simulink library "IO"  (R2024a)
settings: Solver=VariableStepAuto  StartTime=0.0  StopTime=10.0  RelTol=1e-3
values from neighbouring files (symbols this model uses):
  ADCBits = 12.0    [IO.sldd]
  DigitalPolarity : value not decoded    [IO.sldd]
  Vref = 5.0    [IO.sldd]
undefined symbols (not defined in the file or in its folder): Bridge, dt, enum2Raptor, H, raptor_xcp_function
libraries: Raptor_lib x118, Utilities x27, Cooling x1
(part 3 of 4)

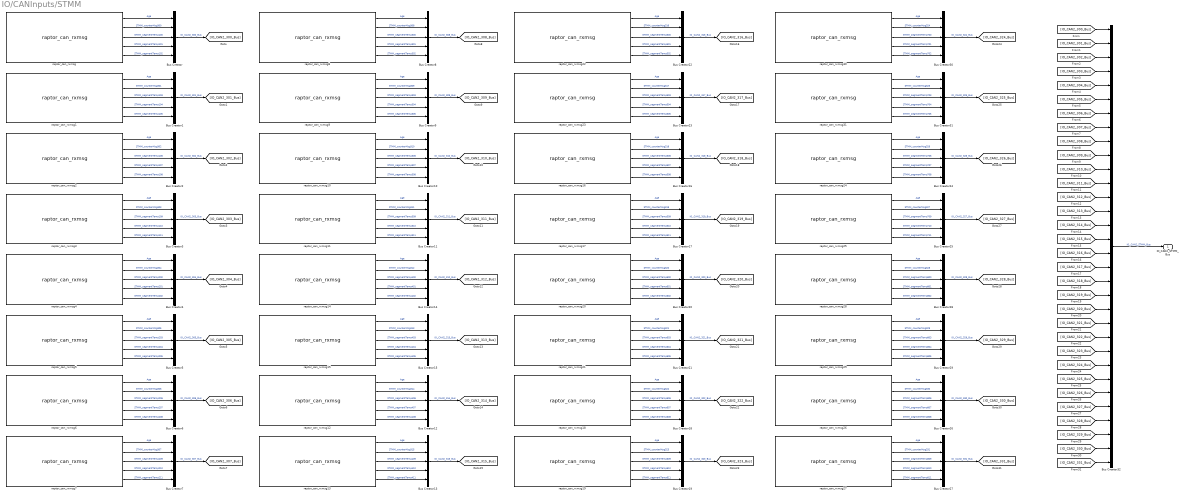
== system IO/CANInputs/STMM ==
  Bus Creator{,1..31} (32 alike) : BusCreator  Inputs=5
  Bus Creator32 : BusCreator  Inputs=32
  raptor_can_rxmsg : Raptor_lib/CAN/raptor_can_rxmsg  canDefinition=struct('dbcFile', 'raptor_CAN2.dbc','message', 'STMM_300','comment', '','signals', {{'STMM_counterMsg300','STMM_segmentTemp100','STMM_segmentTemp101','STMM_segmentTemp102'}},'enabled', [ 1 1 1 1;],'scaled', [ 1 1 1 1;],'canBus', '''CAN2''','messageID', [ 300;],'idMask', [ 536870911;],'payloadMask', [],'payloadValue', [],'period', [ 0;],'mailbox', '''''','queueSize', [ 1;],'label', [ 1;],'ver', [ 2;],'showID', [ 0;],'showRaw', [ 0;],'showRawMsg', [ 0;],'useStartVals', [ 0;],'extendedId', [ 0;],'showAge', [ 1;],'useSimFunc', [ 0;],'sim_func_name', '''''','fill', [ 0;],'editID', [ 0;],'signalOrder', [ 1;],'signalAscDes', [ 1;],'msgLength', [ 8;])  canBus='CAN2'  mailbox=''  payloadMask=[]  payloadValue=[]  idMask=hex2dec('1FFFFFFF')  queueSize=1  showID=0  label=1  fill=0  id=300  showRaw=0  showAge=1  signalOrder=1  signalInfo={{struct('Name', 'STMM_counterMsg300','StartBit', [ 0;],'SignalSize', [ 4;],'ByteOrder', 'LittleEndian','ValueType', 'UNSIGNED','Class', 'uint8','Signed', [ 0;],'Factor', [ 1;],'Offset', [ 0;],'Min', [ 0;],'Max', [ 15;],'Units', '','StartVal', [ 0;],'Comment', 'Counter Message 300','Multiplexed', [ 0;],'Multiplexor', [ 0;],'MultiplexMode_Min', [],'MultiplexMode_Max', []),struct('Name', 'STMM_segmentTemp100','StartBit', [ 16;],'SignalSize', [ 16;],'ByteOrder', 'LittleEndian','ValueType', 'SIGNED','Class', 'int16','Signed', [ 1;],'Factor', [ 0.1;],'Offset', [ 0;],'Min', [ -5;],'Max', [ 120;],'Units', 'degC','StartVal', [ 0;],'Comment', 'Segment 1 module 0','Multiplexed', [ 0;],'Multiplexor', [ 0;],'MultiplexMode_Min', [],'MultiplexMode_Max', []),struct('Name', 'STMM_segmentTemp101','StartBit', [ 32;],'SignalSize', [ 16;],'ByteOrder', 'LittleEndian','ValueType', 'SIGNED','Class', 'int16','Signed', [ 1;],'Factor', [ 0.1;],'Offset', [ 0;],'Min', [ -5;],'Max', [ 120;],'Units', 'degC','StartVal', [ 0;],'Comment', 'Segment 1 module 1','Multiplexed', [ 0;],'Multiplexor', [ 0;],'MultiplexMode_Min', [],'MultiplexMode_Max', []),struct('Name', 'STMM_segmentTemp102','StartBit', [ 48;],'SignalSize', [ 16;],'ByteOrder', 'LittleEndian','ValueType', 'SIGNED','Class', 'int16','Signed', [ 1;],'Factor', [ 0.1;],'Offset', [ 0;],'Min', [ -5;],'Max', [ 120;],'Units', 'degC','StartVal', [ 0;],'Comment', 'Segment 1 module 2','Multiplexed', [ 0;],'Multiplexor', [ 0;],'MultiplexMode_Min', [],'MultiplexMode_Max', [])}}  showRawMsg=0  useSimFunc=0  sim_func_name=''  useStartVals=0  extendedId=0
      settings: SourceProductName=Raptor
  raptor_can_rxmsg1 : Raptor_lib/CAN/raptor_can_rxmsg  canDefinition=struct('dbcFile', 'raptor_CAN2.dbc','message', 'STMM_301','comment', '','signals', {{'STMM_counterMsg301','STMM_segmentTemp103','STMM_segmentTemp104','STMM_segmentTemp105'}},'enabled', [ 1 1 1 1;],'scaled', [ 1 1 1 1;],'canBus', '''CAN2''','messageID', [ 301;],'idMask', [ 536870911;],'payloadMask', [],'payloadValue', [],'period', [ 0;],'mailbox', '''''','queueSize', [ 1;],'label', [ 1;],'ver', [ 2;],'showID', [ 0;],'showRaw', [ 0;],'showRawMsg', [ 0;],'useStartVals', [ 0;],'extendedId', [ 0;],'showAge', [ 1;],'useSimFunc', [ 0;],'sim_func_name', '''''','fill', [ 0;],'editID', [ 0;],'signalOrder', [ 1;],'signalAscDes', [ 1;],'msgLength', [ 8;])  canBus='CAN2'  mailbox=''  payloadMask=[]  payloadValue=[]  idMask=hex2dec('1FFFFFFF')  queueSize=1  showID=0  label=1  fill=0  id=301  showRaw=0  showAge=1  signalOrder=1  signalInfo={{struct('Name', 'STMM_counterMsg301','StartBit', [ 0;],'SignalSize', [ 4;],'ByteOrder', 'LittleEndian','ValueType', 'UNSIGNED','Class', 'uint8','Signed', [ 0;],'Factor', [ 1;],'Offset', [ 0;],'Min', [ 0;],'Max', [ 15;],'Units', '','StartVal', [ 0;],'Comment', 'Counter Message 301','Multiplexed', [ 0;],'Multiplexor', [ 0;],'MultiplexMode_Min', [],'MultiplexMode_Max', []),struct('Name', 'STMM_segmentTemp103','StartBit', [ 16;],'SignalSize', [ 16;],'ByteOrder', 'LittleEndian','ValueType', 'SIGNED','Class', 'int16','Signed', [ 1;],'Factor', [ 0.1;],'Offset', [ 0;],'Min', [ -5;],'Max', [ 120;],'Units', 'degC','StartVal', [ 0;],'Comment', 'Segment 1 module 3','Multiplexed', [ 0;],'Multiplexor', [ 0;],'MultiplexMode_Min', [],'MultiplexMode_Max', []),struct('Name', 'STMM_segmentTemp104','StartBit', [ 32;],'SignalSize', [ 16;],'ByteOrder', 'LittleEndian','ValueType', 'SIGNED','Class', 'int16','Signed', [ 1;],'Factor', [ 0.1;],'Offset', [ 0;],'Min', [ -5;],'Max', [ 120;],'Units', 'degC','StartVal', [ 0;],'Comment', 'Segment 1 module 4','Multiplexed', [ 0;],'Multiplexor', [ 0;],'MultiplexMode_Min', [],'MultiplexMode_Max', []),struct('Name', 'STMM_segmentTemp105','StartBit', [ 48;],'SignalSize', [ 16;],'ByteOrder', 'LittleEndian','ValueType', 'SIGNED','Class', 'int16','Signed', [ 1;],'Factor', [ 0.1;],'Offset', [ 0;],'Min', [ -5;],'Max', [ 120;],'Units', 'degC','StartVal', [ 0;],'Comment', 'Segment 1 module 5','Multiplexed', [ 0;],'Multiplexor', [ 0;],'MultiplexMode_Min', [],'MultiplexMode_Max', [])}}  showRawMsg=0  useSimFunc=0  sim_func_name=''  useStartVals=0  extendedId=0
      settings: SourceProductName=Raptor
  raptor_can_rxmsg10 : Raptor_lib/CAN/raptor_can_rxmsg  canDefinition=struct('dbcFile', 'raptor_CAN2.dbc','message', 'STMM_310','comment', '','signals', {{'STMM_counterMsg310','STMM_segmentTemp306','STMM_segmentTemp307','STMM_segmentTemp308'}},'enabled', [ 1 1 1 1;],'scaled', [ 1 1 1 1;],'canBus', '''CAN2''','messageID', [ 310;],'idMask', [ 536870911;],'payloadMask', [],'payloadValue', [],'period', [ 0;],'mailbox', '''''','queueSize', [ 1;],'label', [ 1;],'ver', [ 2;],'showID', [ 0;],'showRaw', [ 0;],'showRawMsg', [ 0;],'useStartVals', [ 0;],'extendedId', [ 0;],'showAge', [ 1;],'useSimFunc', [ 0;],'sim_func_name', '''''','fill', [ 0;],'editID', [ 0;],'signalOrder', [ 1;],'signalAscDes', [ 1;],'msgLength', [ 8;])  canBus='CAN2'  mailbox=''  payloadMask=[]  payloadValue=[]  idMask=hex2dec('1FFFFFFF')  queueSize=1  showID=0  label=1  fill=0  id=310  showRaw=0  showAge=1  signalOrder=1  signalInfo={{struct('Name', 'STMM_counterMsg310','StartBit', [ 0;],'SignalSize', [ 4;],'ByteOrder', 'LittleEndian','ValueType', 'UNSIGNED','Class', 'uint8','Signed', [ 0;],'Factor', [ 1;],'Offset', [ 0;],'Min', [ 0;],'Max', [ 15;],'Units', '','StartVal', [ 0;],'Comment', 'Counter Message 310','Multiplexed', [ 0;],'Multiplexor', [ 0;],'MultiplexMode_Min', [],'MultiplexMode_Max', []),struct('Name', 'STMM_segmentTemp306','StartBit', [ 16;],'SignalSize', [ 16;],'ByteOrder', 'LittleEndian','ValueType', 'SIGNED','Class', 'int16','Signed', [ 1;],'Factor', [ 0.1;],'Offset', [ 0;],'Min', [ -5;],'Max', [ 120;],'Units', 'degC','StartVal', [ 0;],'Comment', 'Segment 3 module 6','Multiplexed', [ 0;],'Multiplexor', [ 0;],'MultiplexMode_Min', [],'MultiplexMode_Max', []),struct('Name', 'STMM_segmentTemp307','StartBit', [ 32;],'SignalSize', [ 16;],'ByteOrder', 'LittleEndian','ValueType', 'SIGNED','Class', 'int16','Signed', [ 1;],'Factor', [ 0.1;],'Offset', [ 0;],'Min', [ -5;],'Max', [ 120;],'Units', 'degC','StartVal', [ 0;],'Comment', 'Segment 3 module 7','Multiplexed', [ 0;],'Multiplexor', [ 0;],'MultiplexMode_Min', [],'MultiplexMode_Max', []),struct('Name', 'STMM_segmentTemp308','StartBit', [ 48;],'SignalSize', [ 16;],'ByteOrder', 'LittleEndian','ValueType', 'SIGNED','Class', 'int16','Signed', [ 1;],'Factor', [ 0.1;],'Offset', [ 0;],'Min', [ -5;],'Max', [ 120;],'Units', 'degC','StartVal', [ 0;],'Comment', 'Segment 3 module 8','Multiplexed', [ 0;],'Multiplexor', [ 0;],'MultiplexMode_Min', [],'MultiplexMode_Max', [])}}  showRawMsg=0  useSimFunc=0  sim_func_name=''  useStartVals=0  extendedId=0
      settings: SourceProductName=Raptor
  raptor_can_rxmsg11 : Raptor_lib/CAN/raptor_can_rxmsg  canDefinition=struct('dbcFile', 'raptor_CAN2.dbc','message', 'STMM_311','comment', '','signals', {{'STMM_counterMsg311','STMM_segmentTemp309','STMM_segmentTemp310','STMM_segmentTemp311'}},'enabled', [ 1 1 1 1;],'scaled', [ 1 1 1 1;],'canBus', '''CAN2''','messageID', [ 311;],'idMask', [ 536870911;],'payloadMask', [],'payloadValue', [],'period', [ 0;],'mailbox', '''''','queueSize', [ 1;],'label', [ 1;],'ver', [ 2;],'showID', [ 0;],'showRaw', [ 0;],'showRawMsg', [ 0;],'useStartVals', [ 0;],'extendedId', [ 0;],'showAge', [ 1;],'useSimFunc', [ 0;],'sim_func_name', '''''','fill', [ 0;],'editID', [ 0;],'signalOrder', [ 1;],'signalAscDes', [ 1;],'msgLength', [ 8;])  canBus='CAN2'  mailbox=''  payloadMask=[]  payloadValue=[]  idMask=hex2dec('1FFFFFFF')  queueSize=1  showID=0  label=1  fill=0  id=311  showRaw=0  showAge=1  signalOrder=1  signalInfo={{struct('Name', 'STMM_segmentTemp311','StartBit', [ 48;],'SignalSize', [ 16;],'ByteOrder', 'LittleEndian','ValueType', 'SIGNED','Class', 'int16','Signed', [ 1;],'Factor', [ 0.1;],'Offset', [ 0;],'Min', [ -5;],'Max', [ 120;],'Units', 'degC','StartVal', [ 0;],'Comment', 'Segment 3 module 11','Multiplexed', [ 0;],'Multiplexor', [ 0;],'MultiplexMode_Min', [],'MultiplexMode_Max', []),struct('Name', 'STMM_segmentTemp310','StartBit', [ 32;],'SignalSize', [ 16;],'ByteOrder', 'LittleEndian','ValueType', 'SIGNED','Class', 'int16','Signed', [ 1;],'Factor', [ 0.1;],'Offset', [ 0;],'Min', [ -5;],'Max', [ 120;],'Units', 'degC','StartVal', [ 0;],'Comment', 'Segment 3 module 10','Multiplexed', [ 0;],'Multiplexor', [ 0;],'MultiplexMode_Min', [],'MultiplexMode_Max', []),struct('Name', 'STMM_segmentTemp309','StartBit', [ 16;],'SignalSize', [ 16;],'ByteOrder', 'LittleEndian','ValueType', 'SIGNED','Class', 'int16','Signed', [ 1;],'Factor', [ 0.1;],'Offset', [ 0;],'Min', [ -5;],'Max', [ 120;],'Units', 'degC','StartVal', [ 0;],'Comment', 'Segment 3 module 9','Multiplexed', [ 0;],'Multiplexor', [ 0;],'MultiplexMode_Min', [],'MultiplexMode_Max', []),struct('Name', 'STMM_counterMsg311','StartBit', [ 0;],'SignalSize', [ 4;],'ByteOrder', 'LittleEndian','ValueType', 'UNSIGNED','Class', 'uint8','Signed', [ 0;],'Factor', [ 1;],'Offset', [ 0;],'Min', [ 0;],'Max', [ 15;],'Units', '','StartVal', [ 0;],'Comment', 'Counter Message 311','Multiplexed', [ 0;],'Multiplexor', [ 0;],'MultiplexMode_Min', [],'MultiplexMode_Max', [])}}  showRawMsg=0  useSimFunc=0  sim_func_name=''  useStartVals=0  extendedId=0
      settings: SourceProductName=Raptor
  raptor_can_rxmsg12 : Raptor_lib/CAN/raptor_can_rxmsg  canDefinition=struct('dbcFile', 'raptor_CAN2.dbc','message', 'STMM_314','comment', '','signals', {{'STMM_counterMsg314','STMM_segmentTemp406','STMM_segmentTemp407','STMM_segmentTemp408'}},'enabled', [ 1 1 1 1;],'scaled', [ 1 1 1 1;],'canBus', '''CAN2''','messageID', [ 314;],'idMask', [ 536870911;],'payloadMask', [],'payloadValue', [],'period', [ 0;],'mailbox', '''''','queueSize', [ 1;],'label', [ 1;],'ver', [ 2;],'showID', [ 0;],'showRaw', [ 0;],'showRawMsg', [ 0;],'useStartVals', [ 0;],'extendedId', [ 0;],'showAge', [ 1;],'useSimFunc', [ 0;],'sim_func_name', '''''','fill', [ 0;],'editID', [ 0;],'signalOrder', [ 1;],'signalAscDes', [ 1;],'msgLength', [ 8;])  canBus='CAN2'  mailbox=''  payloadMask=[]  payloadValue=[]  idMask=hex2dec('1FFFFFFF')  queueSize=1  showID=0  label=1  fill=0  id=314  showRaw=0  showAge=1  signalOrder=1  signalInfo={{struct('Name', 'STMM_segmentTemp408','StartBit', [ 48;],'SignalSize', [ 16;],'ByteOrder', 'LittleEndian','ValueType', 'SIGNED','Class', 'int16','Signed', [ 1;],'Factor', [ 0.1;],'Offset', [ 0;],'Min', [ -5;],'Max', [ 120;],'Units', 'degC','StartVal', [ 0;],'Comment', 'Segment 4 module 8','Multiplexed', [ 0;],'Multiplexor', [ 0;],'MultiplexMode_Min', [],'MultiplexMode_Max', []),struct('Name', 'STMM_segmentTemp407','StartBit', [ 32;],'SignalSize', [ 16;],'ByteOrder', 'LittleEndian','ValueType', 'SIGNED','Class', 'int16','Signed', [ 1;],'Factor', [ 0.1;],'Offset', [ 0;],'Min', [ -5;],'Max', [ 120;],'Units', 'degC','StartVal', [ 0;],'Comment', 'Segment 4 module 7','Multiplexed', [ 0;],'Multiplexor', [ 0;],'MultiplexMode_Min', [],'MultiplexMode_Max', []),struct('Name', 'STMM_segmentTemp406','StartBit', [ 16;],'SignalSize', [ 16;],'ByteOrder', 'LittleEndian','ValueType', 'SIGNED','Class', 'int16','Signed', [ 1;],'Factor', [ 0.1;],'Offset', [ 0;],'Min', [ -5;],'Max', [ 120;],'Units', 'degC','StartVal', [ 0;],'Comment', 'Segment 4 module 6','Multiplexed', [ 0;],'Multiplexor', [ 0;],'MultiplexMode_Min', [],'MultiplexMode_Max', []),struct('Name', 'STMM_counterMsg314','StartBit', [ 0;],'SignalSize', [ 4;],'ByteOrder', 'LittleEndian','ValueType', 'UNSIGNED','Class', 'uint8','Signed', [ 0;],'Factor', [ 1;],'Offset', [ 0;],'Min', [ 0;],'Max', [ 15;],'Units', '','StartVal', [ 0;],'Comment', 'Counter Message 314','Multiplexed', [ 0;],'Multiplexor', [ 0;],'MultiplexMode_Min', [],'MultiplexMode_Max', [])}}  showRawMsg=0  useSimFunc=0  sim_func_name=''  useStartVals=0  extendedId=0
      settings: SourceProductName=Raptor
  raptor_can_rxmsg13 : Raptor_lib/CAN/raptor_can_rxmsg  canDefinition=struct('dbcFile', 'raptor_CAN2.dbc','message', 'STMM_315','comment', '','signals', {{'STMM_counterMsg315','STMM_segmentTemp409','STMM_segmentTemp410','STMM_segmentTemp411'}},'enabled', [ 1 1 1 1;],'scaled', [ 1 1 1 1;],'canBus', '''CAN2''','messageID', [ 315;],'idMask', [ 536870911;],'payloadMask', [],'payloadValue', [],'period', [ 0;],'mailbox', '''''','queueSize', [ 1;],'label', [ 1;],'ver', [ 2;],'showID', [ 0;],'showRaw', [ 0;],'showRawMsg', [ 0;],'useStartVals', [ 0;],'extendedId', [ 0;],'showAge', [ 1;],'useSimFunc', [ 0;],'sim_func_name', '''''','fill', [ 0;],'editID', [ 0;],'signalOrder', [ 1;],'signalAscDes', [ 1;],'msgLength', [ 8;])  canBus='CAN2'  mailbox=''  payloadMask=[]  payloadValue=[]  idMask=hex2dec('1FFFFFFF')  queueSize=1  showID=0  label=1  fill=0  id=315  showRaw=0  showAge=1  signalOrder=1  signalInfo={{struct('Name', 'STMM_segmentTemp411','StartBit', [ 48;],'SignalSize', [ 16;],'ByteOrder', 'LittleEndian','ValueType', 'SIGNED','Class', 'int16','Signed', [ 1;],'Factor', [ 0.1;],'Offset', [ 0;],'Min', [ -5;],'Max', [ 120;],'Units', 'degC','StartVal', [ 0;],'Comment', 'Segment 4 module 11','Multiplexed', [ 0;],'Multiplexor', [ 0;],'MultiplexMode_Min', [],'MultiplexMode_Max', []),struct('Name', 'STMM_segmentTemp410','StartBit', [ 32;],'SignalSize', [ 16;],'ByteOrder', 'LittleEndian','ValueType', 'SIGNED','Class', 'int16','Signed', [ 1;],'Factor', [ 0.1;],'Offset', [ 0;],'Min', [ -5;],'Max', [ 120;],'Units', 'degC','StartVal', [ 0;],'Comment', 'Segment 4 module 10','Multiplexed', [ 0;],'Multiplexor', [ 0;],'MultiplexMode_Min', [],'MultiplexMode_Max', []),struct('Name', 'STMM_segmentTemp409','StartBit', [ 16;],'SignalSize', [ 16;],'ByteOrder', 'LittleEndian','ValueType', 'SIGNED','Class', 'int16','Signed', [ 1;],'Factor', [ 0.1;],'Offset', [ 0;],'Min', [ -5;],'Max', [ 120;],'Units', 'degC','StartVal', [ 0;],'Comment', 'Segment 4 module 9','Multiplexed', [ 0;],'Multiplexor', [ 0;],'MultiplexMode_Min', [],'MultiplexMode_Max', []),struct('Name', 'STMM_counterMsg315','StartBit', [ 0;],'SignalSize', [ 4;],'ByteOrder', 'LittleEndian','ValueType', 'UNSIGNED','Class', 'uint8','Signed', [ 0;],'Factor', [ 1;],'Offset', [ 0;],'Min', [ 0;],'Max', [ 15;],'Units', '','StartVal', [ 0;],'Comment', 'Counter Message 315','Multiplexed', [ 0;],'Multiplexor', [ 0;],'MultiplexMode_Min', [],'MultiplexMode_Max', [])}}  showRawMsg=0  useSimFunc=0  sim_func_name=''  useStartVals=0  extendedId=0
      settings: SourceProductName=Raptor
  raptor_can_rxmsg14 : Raptor_lib/CAN/raptor_can_rxmsg  canDefinition=struct('dbcFile', 'raptor_CAN2.dbc','message', 'STMM_312','comment', '','signals', {{'STMM_counterMsg312','STMM_segmentTemp400','STMM_segmentTemp401','STMM_segmentTemp402'}},'enabled', [ 1 1 1 1;],'scaled', [ 1 1 1 1;],'canBus', '''CAN2''','messageID', [ 312;],'idMask', [ 536870911;],'payloadMask', [],'payloadValue', [],'period', [ 0;],'mailbox', '''''','queueSize', [ 1;],'label', [ 1;],'ver', [ 2;],'showID', [ 0;],'showRaw', [ 0;],'showRawMsg', [ 0;],'useStartVals', [ 0;],'extendedId', [ 0;],'showAge', [ 1;],'useSimFunc', [ 0;],'sim_func_name', '''''','fill', [ 0;],'editID', [ 0;],'signalOrder', [ 1;],'signalAscDes', [ 1;],'msgLength', [ 8;])  canBus='CAN2'  mailbox=''  payloadMask=[]  payloadValue=[]  idMask=hex2dec('1FFFFFFF')  queueSize=1  showID=0  label=1  fill=0  id=312  showRaw=0  showAge=1  signalOrder=1  signalInfo={{struct('Name', 'STMM_segmentTemp402','StartBit', [ 48;],'SignalSize', [ 16;],'ByteOrder', 'LittleEndian','ValueType', 'SIGNED','Class', 'int16','Signed', [ 1;],'Factor', [ 0.1;],'Offset', [ 0;],'Min', [ -5;],'Max', [ 120;],'Units', 'degC','StartVal', [ 0;],'Comment', 'Segment 4 module 2','Multiplexed', [ 0;],'Multiplexor', [ 0;],'MultiplexMode_Min', [],'MultiplexMode_Max', []),struct('Name', 'STMM_segmentTemp401','StartBit', [ 32;],'SignalSize', [ 16;],'ByteOrder', 'LittleEndian','ValueType', 'SIGNED','Class', 'int16','Signed', [ 1;],'Factor', [ 0.1;],'Offset', [ 0;],'Min', [ -5;],'Max', [ 120;],'Units', 'degC','StartVal', [ 0;],'Comment', 'Segment 4 module 1','Multiplexed', [ 0;],'Multiplexor', [ 0;],'MultiplexMode_Min', [],'MultiplexMode_Max', []),struct('Name', 'STMM_segmentTemp400','StartBit', [ 16;],'SignalSize', [ 16;],'ByteOrder', 'LittleEndian','ValueType', 'SIGNED','Class', 'int16','Signed', [ 1;],'Factor', [ 0.1;],'Offset', [ 0;],'Min', [ -5;],'Max', [ 120;],'Units', 'degC','StartVal', [ 0;],'Comment', 'Segment 4 module 0','Multiplexed', [ 0;],'Multiplexor', [ 0;],'MultiplexMode_Min', [],'MultiplexMode_Max', []),struct('Name', 'STMM_counterMsg312','StartBit', [ 0;],'SignalSize', [ 4;],'ByteOrder', 'LittleEndian','ValueType', 'UNSIGNED','Class', 'uint8','Signed', [ 0;],'Factor', [ 1;],'Offset', [ 0;],'Min', [ 0;],'Max', [ 15;],'Units', '','StartVal', [ 0;],'Comment', 'Counter Message 312','Multiplexed', [ 0;],'Multiplexor', [ 0;],'MultiplexMode_Min', [],'MultiplexMode_Max', [])}}  showRawMsg=0  useSimFunc=0  sim_func_name=''  useStartVals=0  extendedId=0
      settings: SourceProductName=Raptor
  raptor_can_rxmsg15 : Raptor_lib/CAN/raptor_can_rxmsg  canDefinition=struct('dbcFile', 'raptor_CAN2.dbc','message', 'STMM_313','comment', '','signals', {{'STMM_counterMsg313','STMM_segmentTemp403','STMM_segmentTemp404','STMM_segmentTemp405'}},'enabled', [ 1 1 1 1;],'scaled', [ 1 1 1 1;],'canBus', '''CAN2''','messageID', [ 313;],'idMask', [ 536870911;],'payloadMask', [],'payloadValue', [],'period', [ 0;],'mailbox', '''''','queueSize', [ 1;],'label', [ 1;],'ver', [ 2;],'showID', [ 0;],'showRaw', [ 0;],'showRawMsg', [ 0;],'useStartVals', [ 0;],'extendedId', [ 0;],'showAge', [ 1;],'useSimFunc', [ 0;],'sim_func_name', '''''','fill', [ 0;],'editID', [ 0;],'signalOrder', [ 1;],'signalAscDes', [ 1;],'msgLength', [ 8;])  canBus='CAN2'  mailbox=''  payloadMask=[]  payloadValue=[]  idMask=hex2dec('1FFFFFFF')  queueSize=1  showID=0  label=1  fill=0  id=313  showRaw=0  showAge=1  signalOrder=1  signalInfo={{struct('Name', 'STMM_segmentTemp405','StartBit', [ 48;],'SignalSize', [ 16;],'ByteOrder', 'LittleEndian','ValueType', 'SIGNED','Class', 'int16','Signed', [ 1;],'Factor', [ 0.1;],'Offset', [ 0;],'Min', [ -5;],'Max', [ 120;],'Units', 'degC','StartVal', [ 0;],'Comment', 'Segment 4 module 5','Multiplexed', [ 0;],'Multiplexor', [ 0;],'MultiplexMode_Min', [],'MultiplexMode_Max', []),struct('Name', 'STMM_segmentTemp404','StartBit', [ 32;],'SignalSize', [ 16;],'ByteOrder', 'LittleEndian','ValueType', 'SIGNED','Class', 'int16','Signed', [ 1;],'Factor', [ 0.1;],'Offset', [ 0;],'Min', [ -5;],'Max', [ 120;],'Units', 'degC','StartVal', [ 0;],'Comment', 'Segment 4 module 4','Multiplexed', [ 0;],'Multiplexor', [ 0;],'MultiplexMode_Min', [],'MultiplexMode_Max', []),struct('Name', 'STMM_segmentTemp403','StartBit', [ 16;],'SignalSize', [ 16;],'ByteOrder', 'LittleEndian','ValueType', 'SIGNED','Class', 'int16','Signed', [ 1;],'Factor', [ 0.1;],'Offset', [ 0;],'Min', [ -5;],'Max', [ 120;],'Units', 'degC','StartVal', [ 0;],'Comment', 'Segment 4 module 3','Multiplexed', [ 0;],'Multiplexor', [ 0;],'MultiplexMode_Min', [],'MultiplexMode_Max', []),struct('Name', 'STMM_counterMsg313','StartBit', [ 0;],'SignalSize', [ 4;],'ByteOrder', 'LittleEndian','ValueType', 'UNSIGNED','Class', 'uint8','Signed', [ 0;],'Factor', [ 1;],'Offset', [ 0;],'Min', [ 0;],'Max', [ 15;],'Units', '','StartVal', [ 0;],'Comment', 'Counter Message 313','Multiplexed', [ 0;],'Multiplexor', [ 0;],'MultiplexMode_Min', [],'MultiplexMode_Max', [])}}  showRawMsg=0  useSimFunc=0  sim_func_name=''  useStartVals=0  extendedId=0
      settings: SourceProductName=Raptor
  raptor_can_rxmsg16 : Raptor_lib/CAN/raptor_can_rxmsg  canDefinition=struct('dbcFile', 'raptor_CAN2.dbc','message', 'STMM_318','comment', '','signals', {{'STMM_counterMsg318','STMM_segmentTemp506','STMM_segmentTemp507','STMM_segmentTemp508'}},'enabled', [ 1 1 1 1;],'scaled', [ 1 1 1 1;],'canBus', '''CAN2''','messageID', [ 318;],'idMask', [ 536870911;],'payloadMask', [],'payloadValue', [],'period', [ 0;],'mailbox', '''''','queueSize', [ 1;],'label', [ 1;],'ver', [ 2;],'showID', [ 0;],'showRaw', [ 0;],'showRawMsg', [ 0;],'useStartVals', [ 0;],'extendedId', [ 0;],'showAge', [ 1;],'useSimFunc', [ 0;],'sim_func_name', '''''','fill', [ 0;],'editID', [ 0;],'signalOrder', [ 1;],'signalAscDes', [ 1;],'msgLength', [ 8;])  canBus='CAN2'  mailbox=''  payloadMask=[]  payloadValue=[]  idMask=hex2dec('1FFFFFFF')  queueSize=1  showID=0  label=1  fill=0  id=318  showRaw=0  showAge=1  signalOrder=1  signalInfo={{struct('Name', 'STMM_segmentTemp508','StartBit', [ 48;],'SignalSize', [ 16;],'ByteOrder', 'LittleEndian','ValueType', 'SIGNED','Class', 'int16','Signed', [ 1;],'Factor', [ 0.1;],'Offset', [ 0;],'Min', [ -5;],'Max', [ 120;],'Units', 'degC','StartVal', [ 0;],'Comment', 'Segment 5 module 8','Multiplexed', [ 0;],'Multiplexor', [ 0;],'MultiplexMode_Min', [],'MultiplexMode_Max', []),struct('Name', 'STMM_segmentTemp507','StartBit', [ 32;],'SignalSize', [ 16;],'ByteOrder', 'LittleEndian','ValueType', 'SIGNED','Class', 'int16','Signed', [ 1;],'Factor', [ 0.1;],'Offset', [ 0;],'Min', [ -5;],'Max', [ 120;],'Units', 'degC','StartVal', [ 0;],'Comment', 'Segment 5 module 7','Multiplexed', [ 0;],'Multiplexor', [ 0;],'MultiplexMode_Min', [],'MultiplexMode_Max', []),struct('Name', 'STMM_segmentTemp506','StartBit', [ 16;],'SignalSize', [ 16;],'ByteOrder', 'LittleEndian','ValueType', 'SIGNED','Class', 'int16','Signed', [ 1;],'Factor', [ 0.1;],'Offset', [ 0;],'Min', [ -5;],'Max', [ 120;],'Units', 'degC','StartVal', [ 0;],'Comment', 'Segment 5 module 6','Multiplexed', [ 0;],'Multiplexor', [ 0;],'MultiplexMode_Min', [],'MultiplexMode_Max', []),struct('Name', 'STMM_counterMsg318','StartBit', [ 0;],'SignalSize', [ 4;],'ByteOrder', 'LittleEndian','ValueType', 'UNSIGNED','Class', 'uint8','Signed', [ 0;],'Factor', [ 1;],'Offset', [ 0;],'Min', [ 0;],'Max', [ 15;],'Units', '','StartVal', [ 0;],'Comment', 'Counter Message 318','Multiplexed', [ 0;],'Multiplexor', [ 0;],'MultiplexMode_Min', [],'MultiplexMode_Max', [])}}  showRawMsg=0  useSimFunc=0  sim_func_name=''  useStartVals=0  extendedId=0
      settings: SourceProductName=Raptor
  raptor_can_rxmsg17 : Raptor_lib/CAN/raptor_can_rxmsg  canDefinition=struct('dbcFile', 'raptor_CAN2.dbc','message', 'STMM_319','comment', '','signals', {{'STMM_counterMsg319','STMM_segmentTemp509','STMM_segmentTemp510','STMM_segmentTemp511'}},'enabled', [ 1 1 1 1;],'scaled', [ 1 1 1 1;],'canBus', '''CAN2''','messageID', [ 319;],'idMask', [ 536870911;],'payloadMask', [],'payloadValue', [],'period', [ 0;],'mailbox', '''''','queueSize', [ 1;],'label', [ 1;],'ver', [ 2;],'showID', [ 0;],'showRaw', [ 0;],'showRawMsg', [ 0;],'useStartVals', [ 0;],'extendedId', [ 0;],'showAge', [ 1;],'useSimFunc', [ 0;],'sim_func_name', '''''','fill', [ 0;],'editID', [ 0;],'signalOrder', [ 1;],'signalAscDes', [ 1;],'msgLength', [ 8;])  canBus='CAN2'  mailbox=''  payloadMask=[]  payloadValue=[]  idMask=hex2dec('1FFFFFFF')  queueSize=1  showID=0  label=1  fill=0  id=319  showRaw=0  showAge=1  signalOrder=1  signalInfo={{struct('Name', 'STMM_segmentTemp511','StartBit', [ 48;],'SignalSize', [ 16;],'ByteOrder', 'LittleEndian','ValueType', 'SIGNED','Class', 'int16','Signed', [ 1;],'Factor', [ 0.1;],'Offset', [ 0;],'Min', [ -5;],'Max', [ 120;],'Units', 'degC','StartVal', [ 0;],'Comment', 'Segment 5 module 11','Multiplexed', [ 0;],'Multiplexor', [ 0;],'MultiplexMode_Min', [],'MultiplexMode_Max', []),struct('Name', 'STMM_segmentTemp510','StartBit', [ 32;],'SignalSize', [ 16;],'ByteOrder', 'LittleEndian','ValueType', 'SIGNED','Class', 'int16','Signed', [ 1;],'Factor', [ 0.1;],'Offset', [ 0;],'Min', [ -5;],'Max', [ 120;],'Units', 'degC','StartVal', [ 0;],'Comment', 'Segment 5 module 10','Multiplexed', [ 0;],'Multiplexor', [ 0;],'MultiplexMode_Min', [],'MultiplexMode_Max', []),struct('Name', 'STMM_segmentTemp509','StartBit', [ 16;],'SignalSize', [ 16;],'ByteOrder', 'LittleEndian','ValueType', 'SIGNED','Class', 'int16','Signed', [ 1;],'Factor', [ 0.1;],'Offset', [ 0;],'Min', [ -5;],'Max', [ 120;],'Units', 'degC','StartVal', [ 0;],'Comment', 'Segment 5 module 9','Multiplexed', [ 0;],'Multiplexor', [ 0;],'MultiplexMode_Min', [],'MultiplexMode_Max', []),struct('Name', 'STMM_counterMsg319','StartBit', [ 0;],'SignalSize', [ 4;],'ByteOrder', 'LittleEndian','ValueType', 'UNSIGNED','Class', 'uint8','Signed', [ 0;],'Factor', [ 1;],'Offset', [ 0;],'Min', [ 0;],'Max', [ 15;],'Units', '','StartVal', [ 0;],'Comment', 'Counter Message 319','Multiplexed', [ 0;],'Multiplexor', [ 0;],'MultiplexMode_Min', [],'MultiplexMode_Max', [])}}  showRawMsg=0  useSimFunc=0  sim_func_name=''  useStartVals=0  extendedId=0
      settings: SourceProductName=Raptor
  raptor_can_rxmsg18 : Raptor_lib/CAN/raptor_can_rxmsg  canDefinition=struct('dbcFile', 'raptor_CAN2.dbc','message', 'STMM_322','comment', '','signals', {{'STMM_counterMsg322','STMM_segmentTemp606','STMM_segmentTemp607','STMM_segmentTemp608'}},'enabled', [ 1 1 1 1;],'scaled', [ 1 1 1 1;],'canBus', '''CAN2''','messageID', [ 322;],'idMask', [ 536870911;],'payloadMask', [],'payloadValue', [],'period', [ 0;],'mailbox', '''''','queueSize', [ 1;],'label', [ 1;],'ver', [ 2;],'showID', [ 0;],'showRaw', [ 0;],'showRawMsg', [ 0;],'useStartVals', [ 0;],'extendedId', [ 0;],'showAge', [ 1;],'useSimFunc', [ 0;],'sim_func_name', '''''','fill', [ 0;],'editID', [ 0;],'signalOrder', [ 1;],'signalAscDes', [ 1;],'msgLength', [ 8;])  canBus='CAN2'  mailbox=''  payloadMask=[]  payloadValue=[]  idMask=hex2dec('1FFFFFFF')  queueSize=1  showID=0  label=1  fill=0  id=322  showRaw=0  showAge=1  signalOrder=1  signalInfo={{struct('Name', 'STMM_segmentTemp608','StartBit', [ 48;],'SignalSize', [ 16;],'ByteOrder', 'LittleEndian','ValueType', 'SIGNED','Class', 'int16','Signed', [ 1;],'Factor', [ 0.1;],'Offset', [ 0;],'Min', [ -5;],'Max', [ 120;],'Units', 'degC','StartVal', [ 0;],'Comment', 'Segment 6 module 8','Multiplexed', [ 0;],'Multiplexor', [ 0;],'MultiplexMode_Min', [],'MultiplexMode_Max', []),struct('Name', 'STMM_segmentTemp607','StartBit', [ 32;],'SignalSize', [ 16;],'ByteOrder', 'LittleEndian','ValueType', 'SIGNED','Class', 'int16','Signed', [ 1;],'Factor', [ 0.1;],'Offset', [ 0;],'Min', [ -5;],'Max', [ 120;],'Units', 'degC','StartVal', [ 0;],'Comment', 'Segment 6 module 7','Multiplexed', [ 0;],'Multiplexor', [ 0;],'MultiplexMode_Min', [],'MultiplexMode_Max', []),struct('Name', 'STMM_segmentTemp606','StartBit', [ 16;],'SignalSize', [ 16;],'ByteOrder', 'LittleEndian','ValueType', 'SIGNED','Class', 'int16','Signed', [ 1;],'Factor', [ 0.1;],'Offset', [ 0;],'Min', [ -5;],'Max', [ 120;],'Units', 'degC','StartVal', [ 0;],'Comment', 'Segment 6 module 6','Multiplexed', [ 0;],'Multiplexor', [ 0;],'MultiplexMode_Min', [],'MultiplexMode_Max', []),struct('Name', 'STMM_counterMsg322','StartBit', [ 0;],'SignalSize', [ 4;],'ByteOrder', 'LittleEndian','ValueType', 'UNSIGNED','Class', 'uint8','Signed', [ 0;],'Factor', [ 1;],'Offset', [ 0;],'Min', [ 0;],'Max', [ 15;],'Units', '','StartVal', [ 0;],'Comment', 'Counter Message 322','Multiplexed', [ 0;],'Multiplexor', [ 0;],'MultiplexMode_Min', [],'MultiplexMode_Max', [])}}  showRawMsg=0  useSimFunc=0  sim_func_name=''  useStartVals=0  extendedId=0
      settings: SourceProductName=Raptor
  raptor_can_rxmsg19 : Raptor_lib/CAN/raptor_can_rxmsg  canDefinition=struct('dbcFile', 'raptor_CAN2.dbc','message', 'STMM_323','comment', '','signals', {{'STMM_counterMsg323','STMM_segmentTemp609','STMM_segmentTemp610','STMM_segmentTemp611'}},'enabled', [ 1 1 1 1;],'scaled', [ 1 1 1 1;],'canBus', '''CAN2''','messageID', [ 323;],'idMask', [ 536870911;],'payloadMask', [],'payloadValue', [],'period', [ 0;],'mailbox', '''''','queueSize', [ 1;],'label', [ 1;],'ver', [ 2;],'showID', [ 0;],'showRaw', [ 0;],'showRawMsg', [ 0;],'useStartVals', [ 0;],'extendedId', [ 0;],'showAge', [ 1;],'useSimFunc', [ 0;],'sim_func_name', '''''','fill', [ 0;],'editID', [ 0;],'signalOrder', [ 1;],'signalAscDes', [ 1;],'msgLength', [ 8;])  canBus='CAN2'  mailbox=''  payloadMask=[]  payloadValue=[]  idMask=hex2dec('1FFFFFFF')  queueSize=1  showID=0  label=1  fill=0  id=323  showRaw=0  showAge=1  signalOrder=1  signalInfo={{struct('Name', 'STMM_segmentTemp611','StartBit', [ 48;],'SignalSize', [ 16;],'ByteOrder', 'LittleEndian','ValueType', 'SIGNED','Class', 'int16','Signed', [ 1;],'Factor', [ 0.1;],'Offset', [ 0;],'Min', [ -5;],'Max', [ 120;],'Units', 'degC','StartVal', [ 0;],'Comment', 'Segment 6 module 11','Multiplexed', [ 0;],'Multiplexor', [ 0;],'MultiplexMode_Min', [],'MultiplexMode_Max', []),struct('Name', 'STMM_segmentTemp610','StartBit', [ 32;],'SignalSize', [ 16;],'ByteOrder', 'LittleEndian','ValueType', 'SIGNED','Class', 'int16','Signed', [ 1;],'Factor', [ 0.1;],'Offset', [ 0;],'Min', [ -5;],'Max', [ 120;],'Units', 'degC','StartVal', [ 0;],'Comment', 'Segment 6 module 10','Multiplexed', [ 0;],'Multiplexor', [ 0;],'MultiplexMode_Min', [],'MultiplexMode_Max', []),struct('Name', 'STMM_segmentTemp609','StartBit', [ 16;],'SignalSize', [ 16;],'ByteOrder', 'LittleEndian','ValueType', 'SIGNED','Class', 'int16','Signed', [ 1;],'Factor', [ 0.1;],'Offset', [ 0;],'Min', [ -5;],'Max', [ 120;],'Units', 'degC','StartVal', [ 0;],'Comment', 'Segment 6 module 9','Multiplexed', [ 0;],'Multiplexor', [ 0;],'MultiplexMode_Min', [],'MultiplexMode_Max', []),struct('Name', 'STMM_counterMsg323','StartBit', [ 0;],'SignalSize', [ 4;],'ByteOrder', 'LittleEndian','ValueType', 'UNSIGNED','Class', 'uint8','Signed', [ 0;],'Factor', [ 1;],'Offset', [ 0;],'Min', [ 0;],'Max', [ 15;],'Units', '','StartVal', [ 0;],'Comment', 'Counter Message 323','Multiplexed', [ 0;],'Multiplexor', [ 0;],'MultiplexMode_Min', [],'MultiplexMode_Max', [])}}  showRawMsg=0  useSimFunc=0  sim_func_name=''  useStartVals=0  extendedId=0
      settings: SourceProductName=Raptor
  raptor_can_rxmsg2 : Raptor_lib/CAN/raptor_can_rxmsg  canDefinition=struct('dbcFile', 'raptor_CAN2.dbc','message', 'STMM_302','comment', '','signals', {{'STMM_counterMsg302','STMM_segmentTemp106','STMM_segmentTemp107','STMM_segmentTemp108'}},'enabled', [ 1 1 1 1;],'scaled', [ 1 1 1 1;],'canBus', '''CAN2''','messageID', [ 302;],'idMask', [ 536870911;],'payloadMask', [],'payloadValue', [],'period', [ 0;],'mailbox', '''''','queueSize', [ 1;],'label', [ 1;],'ver', [ 2;],'showID', [ 0;],'showRaw', [ 0;],'showRawMsg', [ 0;],'useStartVals', [ 0;],'extendedId', [ 0;],'showAge', [ 1;],'useSimFunc', [ 0;],'sim_func_name', '''''','fill', [ 0;],'editID', [ 0;],'signalOrder', [ 1;],'signalAscDes', [ 1;],'msgLength', [ 8;])  canBus='CAN2'  mailbox=''  payloadMask=[]  payloadValue=[]  idMask=hex2dec('1FFFFFFF')  queueSize=1  showID=0  label=1  fill=0  id=302  showRaw=0  showAge=1  signalOrder=1  signalInfo={{struct('Name', 'STMM_counterMsg302','StartBit', [ 0;],'SignalSize', [ 4;],'ByteOrder', 'LittleEndian','ValueType', 'UNSIGNED','Class', 'uint8','Signed', [ 0;],'Factor', [ 1;],'Offset', [ 0;],'Min', [ 0;],'Max', [ 15;],'Units', '','StartVal', [ 0;],'Comment', 'Counter Message 302','Multiplexed', [ 0;],'Multiplexor', [ 0;],'MultiplexMode_Min', [],'MultiplexMode_Max', []),struct('Name', 'STMM_segmentTemp106','StartBit', [ 16;],'SignalSize', [ 16;],'ByteOrder', 'LittleEndian','ValueType', 'SIGNED','Class', 'int16','Signed', [ 1;],'Factor', [ 0.1;],'Offset', [ 0;],'Min', [ -5;],'Max', [ 120;],'Units', 'degC','StartVal', [ 0;],'Comment', 'Segment 1 module 6','Multiplexed', [ 0;],'Multiplexor', [ 0;],'MultiplexMode_Min', [],'MultiplexMode_Max', []),struct('Name', 'STMM_segmentTemp107','StartBit', [ 32;],'SignalSize', [ 16;],'ByteOrder', 'LittleEndian','ValueType', 'SIGNED','Class', 'int16','Signed', [ 1;],'Factor', [ 0.1;],'Offset', [ 0;],'Min', [ -5;],'Max', [ 120;],'Units', 'degC','StartVal', [ 0;],'Comment', 'Segment 1 module 7','Multiplexed', [ 0;],'Multiplexor', [ 0;],'MultiplexMode_Min', [],'MultiplexMode_Max', []),struct('Name', 'STMM_segmentTemp108','StartBit', [ 48;],'SignalSize', [ 16;],'ByteOrder', 'LittleEndian','ValueType', 'SIGNED','Class', 'int16','Signed', [ 1;],'Factor', [ 0.1;],'Offset', [ 0;],'Min', [ -5;],'Max', [ 120;],'Units', 'degC','StartVal', [ 0;],'Comment', 'Segment 1 module 8','Multiplexed', [ 0;],'Multiplexor', [ 0;],'MultiplexMode_Min', [],'MultiplexMode_Max', [])}}  showRawMsg=0  useSimFunc=0  sim_func_name=''  useStartVals=0  extendedId=0
      settings: SourceProductName=Raptor
  raptor_can_rxmsg20 : Raptor_lib/CAN/raptor_can_rxmsg  canDefinition=struct('dbcFile', 'raptor_CAN2.dbc','message', 'STMM_320','comment', '','signals', {{'STMM_counterMsg320','STMM_segmentTemp600','STMM_segmentTemp601','STMM_segmentTemp602'}},'enabled', [ 1 1 1 1;],'scaled', [ 1 1 1 1;],'canBus', '''CAN2''','messageID', [ 320;],'idMask', [ 536870911;],'payloadMask', [],'payloadValue', [],'period', [ 0;],'mailbox', '''''','queueSize', [ 1;],'label', [ 1;],'ver', [ 2;],'showID', [ 0;],'showRaw', [ 0;],'showRawMsg', [ 0;],'useStartVals', [ 0;],'extendedId', [ 0;],'showAge', [ 1;],'useSimFunc', [ 0;],'sim_func_name', '''''','fill', [ 0;],'editID', [ 0;],'signalOrder', [ 1;],'signalAscDes', [ 1;],'msgLength', [ 8;])  canBus='CAN2'  mailbox=''  payloadMask=[]  payloadValue=[]  idMask=hex2dec('1FFFFFFF')  queueSize=1  showID=0  label=1  fill=0  id=320  showRaw=0  showAge=1  signalOrder=1  signalInfo={{struct('Name', 'STMM_segmentTemp602','StartBit', [ 48;],'SignalSize', [ 16;],'ByteOrder', 'LittleEndian','ValueType', 'SIGNED','Class', 'int16','Signed', [ 1;],'Factor', [ 0.1;],'Offset', [ 0;],'Min', [ -5;],'Max', [ 120;],'Units', 'degC','StartVal', [ 0;],'Comment', 'Segment 6 module 2','Multiplexed', [ 0;],'Multiplexor', [ 0;],'MultiplexMode_Min', [],'MultiplexMode_Max', []),struct('Name', 'STMM_segmentTemp601','StartBit', [ 32;],'SignalSize', [ 16;],'ByteOrder', 'LittleEndian','ValueType', 'SIGNED','Class', 'int16','Signed', [ 1;],'Factor', [ 0.1;],'Offset', [ 0;],'Min', [ -5;],'Max', [ 120;],'Units', 'degC','StartVal', [ 0;],'Comment', 'Segment 6 module 1','Multiplexed', [ 0;],'Multiplexor', [ 0;],'MultiplexMode_Min', [],'MultiplexMode_Max', []),struct('Name', 'STMM_segmentTemp600','StartBit', [ 16;],'SignalSize', [ 16;],'ByteOrder', 'LittleEndian','ValueType', 'SIGNED','Class', 'int16','Signed', [ 1;],'Factor', [ 0.1;],'Offset', [ 0;],'Min', [ -5;],'Max', [ 120;],'Units', 'degC','StartVal', [ 0;],'Comment', 'Segment 6 module 0','Multiplexed', [ 0;],'Multiplexor', [ 0;],'MultiplexMode_Min', [],'MultiplexMode_Max', []),struct('Name', 'STMM_counterMsg320','StartBit', [ 0;],'SignalSize', [ 4;],'ByteOrder', 'LittleEndian','ValueType', 'UNSIGNED','Class', 'uint8','Signed', [ 0;],'Factor', [ 1;],'Offset', [ 0;],'Min', [ 0;],'Max', [ 15;],'Units', '','StartVal', [ 0;],'Comment', 'Counter Message 320','Multiplexed', [ 0;],'Multiplexor', [ 0;],'MultiplexMode_Min', [],'MultiplexMode_Max', [])}}  showRawMsg=0  useSimFunc=0  sim_func_name=''  useStartVals=0  extendedId=0
      settings: SourceProductName=Raptor
  raptor_can_rxmsg21 : Raptor_lib/CAN/raptor_can_rxmsg  canDefinition=struct('dbcFile', 'raptor_CAN2.dbc','message', 'STMM_321','comment', '','signals', {{'STMM_counterMsg321','STMM_segmentTemp603','STMM_segmentTemp604','STMM_segmentTemp605'}},'enabled', [ 1 1 1 1;],'scaled', [ 1 1 1 1;],'canBus', '''CAN2''','messageID', [ 321;],'idMask', [ 536870911;],'payloadMask', [],'payloadValue', [],'period', [ 0;],'mailbox', '''''','queueSize', [ 1;],'label', [ 1;],'ver', [ 2;],'showID', [ 0;],'showRaw', [ 0;],'showRawMsg', [ 0;],'useStartVals', [ 0;],'extendedId', [ 0;],'showAge', [ 1;],'useSimFunc', [ 0;],'sim_func_name', '''''','fill', [ 0;],'editID', [ 0;],'signalOrder', [ 1;],'signalAscDes', [ 1;],'msgLength', [ 8;])  canBus='CAN2'  mailbox=''  payloadMask=[]  payloadValue=[]  idMask=hex2dec('1FFFFFFF')  queueSize=1  showID=0  label=1  fill=0  id=321  showRaw=0  showAge=1  signalOrder=1  signalInfo={{struct('Name', 'STMM_segmentTemp605','StartBit', [ 48;],'SignalSize', [ 16;],'ByteOrder', 'LittleEndian','ValueType', 'SIGNED','Class', 'int16','Signed', [ 1;],'Factor', [ 0.1;],'Offset', [ 0;],'Min', [ -5;],'Max', [ 120;],'Units', 'degC','StartVal', [ 0;],'Comment', 'Segment 6 module 5','Multiplexed', [ 0;],'Multiplexor', [ 0;],'MultiplexMode_Min', [],'MultiplexMode_Max', []),struct('Name', 'STMM_segmentTemp604','StartBit', [ 32;],'SignalSize', [ 16;],'ByteOrder', 'LittleEndian','ValueType', 'SIGNED','Class', 'int16','Signed', [ 1;],'Factor', [ 0.1;],'Offset', [ 0;],'Min', [ -5;],'Max', [ 120;],'Units', 'degC','StartVal', [ 0;],'Comment', 'Segment 6 module 4','Multiplexed', [ 0;],'Multiplexor', [ 0;],'MultiplexMode_Min', [],'MultiplexMode_Max', []),struct('Name', 'STMM_segmentTemp603','StartBit', [ 16;],'SignalSize', [ 16;],'ByteOrder', 'LittleEndian','ValueType', 'SIGNED','Class', 'int16','Signed', [ 1;],'Factor', [ 0.1;],'Offset', [ 0;],'Min', [ -5;],'Max', [ 120;],'Units', 'degC','StartVal', [ 0;],'Comment', 'Segment 6 module 3','Multiplexed', [ 0;],'Multiplexor', [ 0;],'MultiplexMode_Min', [],'MultiplexMode_Max', []),struct('Name', 'STMM_counterMsg321','StartBit', [ 0;],'SignalSize', [ 4;],'ByteOrder', 'LittleEndian','ValueType', 'UNSIGNED','Class', 'uint8','Signed', [ 0;],'Factor', [ 1;],'Offset', [ 0;],'Min', [ 0;],'Max', [ 15;],'Units', '','StartVal', [ 0;],'Comment', 'Counter Message 321','Multiplexed', [ 0;],'Multiplexor', [ 0;],'MultiplexMode_Min', [],'MultiplexMode_Max', [])}}  showRawMsg=0  useSimFunc=0  sim_func_name=''  useStartVals=0  extendedId=0
      settings: SourceProductName=Raptor
  raptor_can_rxmsg22 : Raptor_lib/CAN/raptor_can_rxmsg  canDefinition=struct('dbcFile', 'raptor_CAN2.dbc','message', 'STMM_316','comment', '','signals', {{'STMM_counterMsg316','STMM_segmentTemp500','STMM_segmentTemp501','STMM_segmentTemp502'}},'enabled', [ 1 1 1 1;],'scaled', [ 1 1 1 1;],'canBus', '''CAN2''','messageID', [ 316;],'idMask', [ 536870911;],'payloadMask', [],'payloadValue', [],'period', [ 0;],'mailbox', '''''','queueSize', [ 1;],'label', [ 1;],'ver', [ 2;],'showID', [ 0;],'showRaw', [ 0;],'showRawMsg', [ 0;],'useStartVals', [ 0;],'extendedId', [ 0;],'showAge', [ 1;],'useSimFunc', [ 0;],'sim_func_name', '''''','fill', [ 0;],'editID', [ 0;],'signalOrder', [ 1;],'signalAscDes', [ 1;],'msgLength', [ 8;])  canBus='CAN2'  mailbox=''  payloadMask=[]  payloadValue=[]  idMask=hex2dec('1FFFFFFF')  queueSize=1  showID=0  label=1  fill=0  id=316  showRaw=0  showAge=1  signalOrder=1  signalInfo={{struct('Name', 'STMM_segmentTemp502','StartBit', [ 48;],'SignalSize', [ 16;],'ByteOrder', 'LittleEndian','ValueType', 'SIGNED','Class', 'int16','Signed', [ 1;],'Factor', [ 0.1;],'Offset', [ 0;],'Min', [ -5;],'Max', [ 120;],'Units', 'degC','StartVal', [ 0;],'Comment', 'Segment 5 module 2','Multiplexed', [ 0;],'Multiplexor', [ 0;],'MultiplexMode_Min', [],'MultiplexMode_Max', []),struct('Name', 'STMM_segmentTemp501','StartBit', [ 32;],'SignalSize', [ 16;],'ByteOrder', 'LittleEndian','ValueType', 'SIGNED','Class', 'int16','Signed', [ 1;],'Factor', [ 0.1;],'Offset', [ 0;],'Min', [ -5;],'Max', [ 120;],'Units', 'degC','StartVal', [ 0;],'Comment', 'Segment 5 module 1','Multiplexed', [ 0;],'Multiplexor', [ 0;],'MultiplexMode_Min', [],'MultiplexMode_Max', []),struct('Name', 'STMM_segmentTemp500','StartBit', [ 16;],'SignalSize', [ 16;],'ByteOrder', 'LittleEndian','ValueType', 'SIGNED','Class', 'int16','Signed', [ 1;],'Factor', [ 0.1;],'Offset', [ 0;],'Min', [ -5;],'Max', [ 120;],'Units', 'degC','StartVal', [ 0;],'Comment', 'Segment 5 module 0','Multiplexed', [ 0;],'Multiplexor', [ 0;],'MultiplexMode_Min', [],'MultiplexMode_Max', []),struct('Name', 'STMM_counterMsg316','StartBit', [ 0;],'SignalSize', [ 4;],'ByteOrder', 'LittleEndian','ValueType', 'UNSIGNED','Class', 'uint8','Signed', [ 0;],'Factor', [ 1;],'Offset', [ 0;],'Min', [ 0;],'Max', [ 15;],'Units', '','StartVal', [ 0;],'Comment', 'Counter Message 316','Multiplexed', [ 0;],'Multiplexor', [ 0;],'MultiplexMode_Min', [],'MultiplexMode_Max', [])}}  showRawMsg=0  useSimFunc=0  sim_func_name=''  useStartVals=0  extendedId=0
      settings: SourceProductName=Raptor
  raptor_can_rxmsg23 : Raptor_lib/CAN/raptor_can_rxmsg  canDefinition=struct('dbcFile', 'raptor_CAN2.dbc','message', 'STMM_317','comment', '','signals', {{'STMM_counterMsg317','STMM_segmentTemp503','STMM_segmentTemp504','STMM_segmentTemp505'}},'enabled', [ 1 1 1 1;],'scaled', [ 1 1 1 1;],'canBus', '''CAN2''','messageID', [ 317;],'idMask', [ 536870911;],'payloadMask', [],'payloadValue', [],'period', [ 0;],'mailbox', '''''','queueSize', [ 1;],'label', [ 1;],'ver', [ 2;],'showID', [ 0;],'showRaw', [ 0;],'showRawMsg', [ 0;],'useStartVals', [ 0;],'extendedId', [ 0;],'showAge', [ 1;],'useSimFunc', [ 0;],'sim_func_name', '''''','fill', [ 0;],'editID', [ 0;],'signalOrder', [ 1;],'signalAscDes', [ 1;],'msgLength', [ 8;])  canBus='CAN2'  mailbox=''  payloadMask=[]  payloadValue=[]  idMask=hex2dec('1FFFFFFF')  queueSize=1  showID=0  label=1  fill=0  id=317  showRaw=0  showAge=1  signalOrder=1  signalInfo={{struct('Name', 'STMM_segmentTemp505','StartBit', [ 48;],'SignalSize', [ 16;],'ByteOrder', 'LittleEndian','ValueType', 'SIGNED','Class', 'int16','Signed', [ 1;],'Factor', [ 0.1;],'Offset', [ 0;],'Min', [ -5;],'Max', [ 120;],'Units', 'degC','StartVal', [ 0;],'Comment', 'Segment 5 module 5','Multiplexed', [ 0;],'Multiplexor', [ 0;],'MultiplexMode_Min', [],'MultiplexMode_Max', []),struct('Name', 'STMM_segmentTemp504','StartBit', [ 32;],'SignalSize', [ 16;],'ByteOrder', 'LittleEndian','ValueType', 'SIGNED','Class', 'int16','Signed', [ 1;],'Factor', [ 0.1;],'Offset', [ 0;],'Min', [ -5;],'Max', [ 120;],'Units', 'degC','StartVal', [ 0;],'Comment', 'Segment 5 module 4','Multiplexed', [ 0;],'Multiplexor', [ 0;],'MultiplexMode_Min', [],'MultiplexMode_Max', []),struct('Name', 'STMM_segmentTemp503','StartBit', [ 16;],'SignalSize', [ 16;],'ByteOrder', 'LittleEndian','ValueType', 'SIGNED','Class', 'int16','Signed', [ 1;],'Factor', [ 0.1;],'Offset', [ 0;],'Min', [ -5;],'Max', [ 120;],'Units', 'degC','StartVal', [ 0;],'Comment', 'Segment 5 module 3','Multiplexed', [ 0;],'Multiplexor', [ 0;],'MultiplexMode_Min', [],'MultiplexMode_Max', []),struct('Name', 'STMM_counterMsg317','StartBit', [ 0;],'SignalSize', [ 4;],'ByteOrder', 'LittleEndian','ValueType', 'UNSIGNED','Class', 'uint8','Signed', [ 0;],'Factor', [ 1;],'Offset', [ 0;],'Min', [ 0;],'Max', [ 15;],'Units', '','StartVal', [ 0;],'Comment', 'Counter Message 317','Multiplexed', [ 0;],'Multiplexor', [ 0;],'MultiplexMode_Min', [],'MultiplexMode_Max', [])}}  showRawMsg=0  useSimFunc=0  sim_func_name=''  useStartVals=0  extendedId=0
      settings: SourceProductName=Raptor
  raptor_can_rxmsg24 : Raptor_lib/CAN/raptor_can_rxmsg  canDefinition=struct('dbcFile', 'raptor_CAN2.dbc','message', 'STMM_326','comment', '','signals', {{'STMM_counterMsg326','STMM_segmentTemp706','STMM_segmentTemp707','STMM_segmentTemp708'}},'enabled', [ 1 1 1 1;],'scaled', [ 1 1 1 1;],'canBus', '''CAN2''','messageID', [ 326;],'idMask', [ 536870911;],'payloadMask', [],'payloadValue', [],'period', [ 0;],'mailbox', '''''','queueSize', [ 1;],'label', [ 1;],'ver', [ 2;],'showID', [ 0;],'showRaw', [ 0;],'showRawMsg', [ 0;],'useStartVals', [ 0;],'extendedId', [ 0;],'showAge', [ 1;],'useSimFunc', [ 0;],'sim_func_name', '''''','fill', [ 0;],'editID', [ 0;],'signalOrder', [ 1;],'signalAscDes', [ 1;],'msgLength', [ 8;])  canBus='CAN2'  mailbox=''  payloadMask=[]  payloadValue=[]  idMask=hex2dec('1FFFFFFF')  queueSize=1  showID=0  label=1  fill=0  id=326  showRaw=0  showAge=1  signalOrder=1  signalInfo={{struct('Name', 'STMM_segmentTemp708','StartBit', [ 48;],'SignalSize', [ 16;],'ByteOrder', 'LittleEndian','ValueType', 'SIGNED','Class', 'int16','Signed', [ 1;],'Factor', [ 0.1;],'Offset', [ 0;],'Min', [ -5;],'Max', [ 120;],'Units', 'degC','StartVal', [ 0;],'Comment', 'Segment 7 module 8','Multiplexed', [ 0;],'Multiplexor', [ 0;],'MultiplexMode_Min', [],'MultiplexMode_Max', []),struct('Name', 'STMM_segmentTemp707','StartBit', [ 32;],'SignalSize', [ 16;],'ByteOrder', 'LittleEndian','ValueType', 'SIGNED','Class', 'int16','Signed', [ 1;],'Factor', [ 0.1;],'Offset', [ 0;],'Min', [ -5;],'Max', [ 120;],'Units', 'degC','StartVal', [ 0;],'Comment', 'Segment 7 module 7','Multiplexed', [ 0;],'Multiplexor', [ 0;],'MultiplexMode_Min', [],'MultiplexMode_Max', []),struct('Name', 'STMM_segmentTemp706','StartBit', [ 16;],'SignalSize', [ 16;],'ByteOrder', 'LittleEndian','ValueType', 'SIGNED','Class', 'int16','Signed', [ 1;],'Factor', [ 0.1;],'Offset', [ 0;],'Min', [ -5;],'Max', [ 120;],'Units', 'degC','StartVal', [ 0;],'Comment', 'Segment 7 module 6','Multiplexed', [ 0;],'Multiplexor', [ 0;],'MultiplexMode_Min', [],'MultiplexMode_Max', []),struct('Name', 'STMM_counterMsg326','StartBit', [ 0;],'SignalSize', [ 4;],'ByteOrder', 'LittleEndian','ValueType', 'UNSIGNED','Class', 'uint8','Signed', [ 0;],'Factor', [ 1;],'Offset', [ 0;],'Min', [ 0;],'Max', [ 15;],'Units', '','StartVal', [ 0;],'Comment', 'Counter Message 326','Multiplexed', [ 0;],'Multiplexor', [ 0;],'MultiplexMode_Min', [],'MultiplexMode_Max', [])}}  showRawMsg=0  useSimFunc=0  sim_func_name=''  useStartVals=0  extendedId=0
      settings: SourceProductName=Raptor
  raptor_can_rxmsg25 : Raptor_lib/CAN/raptor_can_rxmsg  canDefinition=struct('dbcFile', 'raptor_CAN2.dbc','message', 'STMM_327','comment', '','signals', {{'STMM_counterMsg327','STMM_segmentTemp709','STMM_segmentTemp710','STMM_segmentTemp711'}},'enabled', [ 1 1 1 1;],'scaled', [ 1 1 1 1;],'canBus', '''CAN2''','messageID', [ 327;],'idMask', [ 536870911;],'payloadMask', [],'payloadValue', [],'period', [ 0;],'mailbox', '''''','queueSize', [ 1;],'label', [ 1;],'ver', [ 2;],'showID', [ 0;],'showRaw', [ 0;],'showRawMsg', [ 0;],'useStartVals', [ 0;],'extendedId', [ 0;],'showAge', [ 1;],'useSimFunc', [ 0;],'sim_func_name', '''''','fill', [ 0;],'editID', [ 0;],'signalOrder', [ 1;],'signalAscDes', [ 1;],'msgLength', [ 8;])  canBus='CAN2'  mailbox=''  payloadMask=[]  payloadValue=[]  idMask=hex2dec('1FFFFFFF')  queueSize=1  showID=0  label=1  fill=0  id=327  showRaw=0  showAge=1  signalOrder=1  signalInfo={{struct('Name', 'STMM_segmentTemp711','StartBit', [ 48;],'SignalSize', [ 16;],'ByteOrder', 'LittleEndian','ValueType', 'SIGNED','Class', 'int16','Signed', [ 1;],'Factor', [ 0.1;],'Offset', [ 0;],'Min', [ -5;],'Max', [ 120;],'Units', 'degC','StartVal', [ 0;],'Comment', 'Segment 7 module 11','Multiplexed', [ 0;],'Multiplexor', [ 0;],'MultiplexMode_Min', [],'MultiplexMode_Max', []),struct('Name', 'STMM_segmentTemp710','StartBit', [ 32;],'SignalSize', [ 16;],'ByteOrder', 'LittleEndian','ValueType', 'SIGNED','Class', 'int16','Signed', [ 1;],'Factor', [ 0.1;],'Offset', [ 0;],'Min', [ -5;],'Max', [ 120;],'Units', 'degC','StartVal', [ 0;],'Comment', 'Segment 7 module 10','Multiplexed', [ 0;],'Multiplexor', [ 0;],'MultiplexMode_Min', [],'MultiplexMode_Max', []),struct('Name', 'STMM_segmentTemp709','StartBit', [ 16;],'SignalSize', [ 16;],'ByteOrder', 'LittleEndian','ValueType', 'SIGNED','Class', 'int16','Signed', [ 1;],'Factor', [ 0.1;],'Offset', [ 0;],'Min', [ -5;],'Max', [ 120;],'Units', 'degC','StartVal', [ 0;],'Comment', 'Segment 7 module 9','Multiplexed', [ 0;],'Multiplexor', [ 0;],'MultiplexMode_Min', [],'MultiplexMode_Max', []),struct('Name', 'STMM_counterMsg327','StartBit', [ 0;],'SignalSize', [ 4;],'ByteOrder', 'LittleEndian','ValueType', 'UNSIGNED','Class', 'uint8','Signed', [ 0;],'Factor', [ 1;],'Offset', [ 0;],'Min', [ 0;],'Max', [ 15;],'Units', '','StartVal', [ 0;],'Comment', 'Counter Message 327','Multiplexed', [ 0;],'Multiplexor', [ 0;],'MultiplexMode_Min', [],'MultiplexMode_Max', [])}}  showRawMsg=0  useSimFunc=0  sim_func_name=''  useStartVals=0  extendedId=0
      settings: SourceProductName=Raptor
  raptor_can_rxmsg26 : Raptor_lib/CAN/raptor_can_rxmsg  canDefinition=struct('dbcFile', 'raptor_CAN2.dbc','message', 'STMM_330','comment', '','signals', {{'STMM_counterMsg330','STMM_segmentTemp806','STMM_segmentTemp807','STMM_segmentTemp808'}},'enabled', [ 1 1 1 1;],'scaled', [ 1 1 1 1;],'canBus', '''CAN2''','messageID', [ 330;],'idMask', [ 536870911;],'payloadMask', [],'payloadValue', [],'period', [ 0;],'mailbox', '''''','queueSize', [ 1;],'label', [ 1;],'ver', [ 2;],'showID', [ 0;],'showRaw', [ 0;],'showRawMsg', [ 0;],'useStartVals', [ 0;],'extendedId', [ 0;],'showAge', [ 1;],'useSimFunc', [ 0;],'sim_func_name', '''''','fill', [ 0;],'editID', [ 0;],'signalOrder', [ 1;],'signalAscDes', [ 1;],'msgLength', [ 8;])  canBus='CAN2'  mailbox=''  payloadMask=[]  payloadValue=[]  idMask=hex2dec('1FFFFFFF')  queueSize=1  showID=0  label=1  fill=0  id=330  showRaw=0  showAge=1  signalOrder=1  signalInfo={{struct('Name', 'STMM_segmentTemp808','StartBit', [ 48;],'SignalSize', [ 16;],'ByteOrder', 'LittleEndian','ValueType', 'SIGNED','Class', 'int16','Signed', [ 1;],'Factor', [ 0.1;],'Offset', [ 0;],'Min', [ -5;],'Max', [ 120;],'Units', 'degC','StartVal', [ 0;],'Comment', 'Segment 8 module 8','Multiplexed', [ 0;],'Multiplexor', [ 0;],'MultiplexMode_Min', [],'MultiplexMode_Max', []),struct('Name', 'STMM_segmentTemp807','StartBit', [ 32;],'SignalSize', [ 16;],'ByteOrder', 'LittleEndian','ValueType', 'SIGNED','Class', 'int16','Signed', [ 1;],'Factor', [ 0.1;],'Offset', [ 0;],'Min', [ -5;],'Max', [ 120;],'Units', 'degC','StartVal', [ 0;],'Comment', 'Segment 8 module 7','Multiplexed', [ 0;],'Multiplexor', [ 0;],'MultiplexMode_Min', [],'MultiplexMode_Max', []),struct('Name', 'STMM_segmentTemp806','StartBit', [ 16;],'SignalSize', [ 16;],'ByteOrder', 'LittleEndian','ValueType', 'SIGNED','Class', 'int16','Signed', [ 1;],'Factor', [ 0.1;],'Offset', [ 0;],'Min', [ -5;],'Max', [ 120;],'Units', 'degC','StartVal', [ 0;],'Comment', 'Segment 8 module 6','Multiplexed', [ 0;],'Multiplexor', [ 0;],'MultiplexMode_Min', [],'MultiplexMode_Max', []),struct('Name', 'STMM_counterMsg330','StartBit', [ 0;],'SignalSize', [ 4;],'ByteOrder', 'LittleEndian','ValueType', 'UNSIGNED','Class', 'uint8','Signed', [ 0;],'Factor', [ 1;],'Offset', [ 0;],'Min', [ 0;],'Max', [ 15;],'Units', '','StartVal', [ 0;],'Comment', 'Counter Message 330','Multiplexed', [ 0;],'Multiplexor', [ 0;],'MultiplexMode_Min', [],'MultiplexMode_Max', [])}}  showRawMsg=0  useSimFunc=0  sim_func_name=''  useStartVals=0  extendedId=0
      settings: SourceProductName=Raptor
  raptor_can_rxmsg27 : Raptor_lib/CAN/raptor_can_rxmsg  canDefinition=struct('dbcFile', 'raptor_CAN2.dbc','message', 'STMM_331','comment', '','signals', {{'STMM_counterMsg331','STMM_segmentTemp809','STMM_segmentTemp810','STMM_segmentTemp811'}},'enabled', [ 1 1 1 1;],'scaled', [ 1 1 1 1;],'canBus', '''CAN2''','messageID', [ 331;],'idMask', [ 536870911;],'payloadMask', [],'payloadValue', [],'period', [ 0;],'mailbox', '''''','queueSize', [ 1;],'label', [ 1;],'ver', [ 2;],'showID', [ 0;],'showRaw', [ 0;],'showRawMsg', [ 0;],'useStartVals', [ 0;],'extendedId', [ 0;],'showAge', [ 1;],'useSimFunc', [ 0;],'sim_func_name', '''''','fill', [ 0;],'editID', [ 0;],'signalOrder', [ 1;],'signalAscDes', [ 1;],'msgLength', [ 8;])  canBus='CAN2'  mailbox=''  payloadMask=[]  payloadValue=[]  idMask=hex2dec('1FFFFFFF')  queueSize=1  showID=0  label=1  fill=0  id=331  showRaw=0  showAge=1  signalOrder=1  signalInfo={{struct('Name', 'STMM_segmentTemp811','StartBit', [ 48;],'SignalSize', [ 16;],'ByteOrder', 'LittleEndian','ValueType', 'SIGNED','Class', 'int16','Signed', [ 1;],'Factor', [ 0.1;],'Offset', [ 0;],'Min', [ -5;],'Max', [ 120;],'Units', 'degC','StartVal', [ 0;],'Comment', 'Segment 8 module 11','Multiplexed', [ 0;],'Multiplexor', [ 0;],'MultiplexMode_Min', [],'MultiplexMode_Max', []),struct('Name', 'STMM_segmentTemp810','StartBit', [ 32;],'SignalSize', [ 16;],'ByteOrder', 'LittleEndian','ValueType', 'SIGNED','Class', 'int16','Signed', [ 1;],'Factor', [ 0.1;],'Offset', [ 0;],'Min', [ -5;],'Max', [ 120;],'Units', 'degC','StartVal', [ 0;],'Comment', 'Segment 8 module 10','Multiplexed', [ 0;],'Multiplexor', [ 0;],'MultiplexMode_Min', [],'MultiplexMode_Max', []),struct('Name', 'STMM_segmentTemp809','StartBit', [ 16;],'SignalSize', [ 16;],'ByteOrder', 'LittleEndian','ValueType', 'SIGNED','Class', 'int16','Signed', [ 1;],'Factor', [ 0.1;],'Offset', [ 0;],'Min', [ -5;],'Max', [ 120;],'Units', 'degC','StartVal', [ 0;],'Comment', 'Segment 8 module 9','Multiplexed', [ 0;],'Multiplexor', [ 0;],'MultiplexMode_Min', [],'MultiplexMode_Max', []),struct('Name', 'STMM_counterMsg331','StartBit', [ 0;],'SignalSize', [ 4;],'ByteOrder', 'LittleEndian','ValueType', 'UNSIGNED','Class', 'uint8','Signed', [ 0;],'Factor', [ 1;],'Offset', [ 0;],'Min', [ 0;],'Max', [ 15;],'Units', '','StartVal', [ 0;],'Comment', 'Counter Message 331','Multiplexed', [ 0;],'Multiplexor', [ 0;],'MultiplexMode_Min', [],'MultiplexMode_Max', [])}}  showRawMsg=0  useSimFunc=0  sim_func_name=''  useStartVals=0  extendedId=0
      settings: SourceProductName=Raptor
  raptor_can_rxmsg28 : Raptor_lib/CAN/raptor_can_rxmsg  canDefinition=struct('dbcFile', 'raptor_CAN2.dbc','message', 'STMM_328','comment', '','signals', {{'STMM_counterMsg328','STMM_segmentTemp800','STMM_segmentTemp801','STMM_segmentTemp802'}},'enabled', [ 1 1 1 1;],'scaled', [ 1 1 1 1;],'canBus', '''CAN2''','messageID', [ 328;],'idMask', [ 536870911;],'payloadMask', [],'payloadValue', [],'period', [ 0;],'mailbox', '''''','queueSize', [ 1;],'label', [ 1;],'ver', [ 2;],'showID', [ 0;],'showRaw', [ 0;],'showRawMsg', [ 0;],'useStartVals', [ 0;],'extendedId', [ 0;],'showAge', [ 1;],'useSimFunc', [ 0;],'sim_func_name', '''''','fill', [ 0;],'editID', [ 0;],'signalOrder', [ 1;],'signalAscDes', [ 1;],'msgLength', [ 8;])  canBus='CAN2'  mailbox=''  payloadMask=[]  payloadValue=[]  idMask=hex2dec('1FFFFFFF')  queueSize=1  showID=0  label=1  fill=0  id=328  showRaw=0  showAge=1  signalOrder=1  signalInfo={{struct('Name', 'STMM_segmentTemp802','StartBit', [ 48;],'SignalSize', [ 16;],'ByteOrder', 'LittleEndian','ValueType', 'SIGNED','Class', 'int16','Signed', [ 1;],'Factor', [ 0.1;],'Offset', [ 0;],'Min', [ -5;],'Max', [ 120;],'Units', 'degC','StartVal', [ 0;],'Comment', 'Segment 8 module 2','Multiplexed', [ 0;],'Multiplexor', [ 0;],'MultiplexMode_Min', [],'MultiplexMode_Max', []),struct('Name', 'STMM_segmentTemp801','StartBit', [ 32;],'SignalSize', [ 16;],'ByteOrder', 'LittleEndian','ValueType', 'SIGNED','Class', 'int16','Signed', [ 1;],'Factor', [ 0.1;],'Offset', [ 0;],'Min', [ -5;],'Max', [ 120;],'Units', 'degC','StartVal', [ 0;],'Comment', 'Segment 8 module 1','Multiplexed', [ 0;],'Multiplexor', [ 0;],'MultiplexMode_Min', [],'MultiplexMode_Max', []),struct('Name', 'STMM_segmentTemp800','StartBit', [ 16;],'SignalSize', [ 16;],'ByteOrder', 'LittleEndian','ValueType', 'SIGNED','Class', 'int16','Signed', [ 1;],'Factor', [ 0.1;],'Offset', [ 0;],'Min', [ -5;],'Max', [ 120;],'Units', 'degC','StartVal', [ 0;],'Comment', 'Segment 8 module 0','Multiplexed', [ 0;],'Multiplexor', [ 0;],'MultiplexMode_Min', [],'MultiplexMode_Max', []),struct('Name', 'STMM_counterMsg328','StartBit', [ 0;],'SignalSize', [ 4;],'ByteOrder', 'LittleEndian','ValueType', 'UNSIGNED','Class', 'uint8','Signed', [ 0;],'Factor', [ 1;],'Offset', [ 0;],'Min', [ 0;],'Max', [ 15;],'Units', '','StartVal', [ 0;],'Comment', 'Counter Message 328','Multiplexed', [ 0;],'Multiplexor', [ 0;],'MultiplexMode_Min', [],'MultiplexMode_Max', [])}}  showRawMsg=0  useSimFunc=0  sim_func_name=''  useStartVals=0  extendedId=0
      settings: SourceProductName=Raptor
  raptor_can_rxmsg29 : Raptor_lib/CAN/raptor_can_rxmsg  canDefinition=struct('dbcFile', 'raptor_CAN2.dbc','message', 'STMM_329','comment', '','signals', {{'STMM_counterMsg329','STMM_segmentTemp803','STMM_segmentTemp804','STMM_segmentTemp805'}},'enabled', [ 1 1 1 1;],'scaled', [ 1 1 1 1;],'canBus', '''CAN2''','messageID', [ 329;],'idMask', [ 536870911;],'payloadMask', [],'payloadValue', [],'period', [ 0;],'mailbox', '''''','queueSize', [ 1;],'label', [ 1;],'ver', [ 2;],'showID', [ 0;],'showRaw', [ 0;],'showRawMsg', [ 0;],'useStartVals', [ 0;],'extendedId', [ 0;],'showAge', [ 1;],'useSimFunc', [ 0;],'sim_func_name', '''''','fill', [ 0;],'editID', [ 0;],'signalOrder', [ 1;],'signalAscDes', [ 1;],'msgLength', [ 8;])  canBus='CAN2'  mailbox=''  payloadMask=[]  payloadValue=[]  idMask=hex2dec('1FFFFFFF')  queueSize=1  showID=0  label=1  fill=0  id=329  showRaw=0  showAge=1  signalOrder=1  signalInfo={{struct('Name', 'STMM_segmentTemp805','StartBit', [ 48;],'SignalSize', [ 16;],'ByteOrder', 'LittleEndian','ValueType', 'SIGNED','Class', 'int16','Signed', [ 1;],'Factor', [ 0.1;],'Offset', [ 0;],'Min', [ -5;],'Max', [ 120;],'Units', 'degC','StartVal', [ 0;],'Comment', 'Segment 8 module 5','Multiplexed', [ 0;],'Multiplexor', [ 0;],'MultiplexMode_Min', [],'MultiplexMode_Max', []),struct('Name', 'STMM_segmentTemp804','StartBit', [ 32;],'SignalSize', [ 16;],'ByteOrder', 'LittleEndian','ValueType', 'SIGNED','Class', 'int16','Signed', [ 1;],'Factor', [ 0.1;],'Offset', [ 0;],'Min', [ -5;],'Max', [ 120;],'Units', 'degC','StartVal', [ 0;],'Comment', 'Segment 8 module 4','Multiplexed', [ 0;],'Multiplexor', [ 0;],'MultiplexMode_Min', [],'MultiplexMode_Max', []),struct('Name', 'STMM_segmentTemp803','StartBit', [ 16;],'SignalSize', [ 16;],'ByteOrder', 'LittleEndian','ValueType', 'SIGNED','Class', 'int16','Signed', [ 1;],'Factor', [ 0.1;],'Offset', [ 0;],'Min', [ -5;],'Max', [ 120;],'Units', 'degC','StartVal', [ 0;],'Comment', 'Segment 8 module 3','Multiplexed', [ 0;],'Multiplexor', [ 0;],'MultiplexMode_Min', [],'MultiplexMode_Max', []),struct('Name', 'STMM_counterMsg329','StartBit', [ 0;],'SignalSize', [ 4;],'ByteOrder', 'LittleEndian','ValueType', 'UNSIGNED','Class', 'uint8','Signed', [ 0;],'Factor', [ 1;],'Offset', [ 0;],'Min', [ 0;],'Max', [ 15;],'Units', '','StartVal', [ 0;],'Comment', 'Counter Message 329','Multiplexed', [ 0;],'Multiplexor', [ 0;],'MultiplexMode_Min', [],'MultiplexMode_Max', [])}}  showRawMsg=0  useSimFunc=0  sim_func_name=''  useStartVals=0  extendedId=0
      settings: SourceProductName=Raptor
  raptor_can_rxmsg3 : Raptor_lib/CAN/raptor_can_rxmsg  canDefinition=struct('dbcFile', 'raptor_CAN2.dbc','message', 'STMM_303','comment', '','signals', {{'STMM_counterMsg303','STMM_segmentTemp109','STMM_segmentTemp110','STMM_segmentTemp111'}},'enabled', [ 1 1 1 1;],'scaled', [ 1 1 1 1;],'canBus', '''CAN2''','messageID', [ 303;],'idMask', [ 536870911;],'payloadMask', [],'payloadValue', [],'period', [ 0;],'mailbox', '''''','queueSize', [ 1;],'label', [ 1;],'ver', [ 2;],'showID', [ 0;],'showRaw', [ 0;],'showRawMsg', [ 0;],'useStartVals', [ 0;],'extendedId', [ 0;],'showAge', [ 1;],'useSimFunc', [ 0;],'sim_func_name', '''''','fill', [ 0;],'editID', [ 0;],'signalOrder', [ 1;],'signalAscDes', [ 1;],'msgLength', [ 8;])  canBus='CAN2'  mailbox=''  payloadMask=[]  payloadValue=[]  idMask=hex2dec('1FFFFFFF')  queueSize=1  showID=0  label=1  fill=0  id=303  showRaw=0  showAge=1  signalOrder=1  signalInfo={{struct('Name', 'STMM_counterMsg303','StartBit', [ 0;],'SignalSize', [ 4;],'ByteOrder', 'LittleEndian','ValueType', 'UNSIGNED','Class', 'uint8','Signed', [ 0;],'Factor', [ 1;],'Offset', [ 0;],'Min', [ 0;],'Max', [ 15;],'Units', '','StartVal', [ 0;],'Comment', 'Counter Message 303','Multiplexed', [ 0;],'Multiplexor', [ 0;],'MultiplexMode_Min', [],'MultiplexMode_Max', []),struct('Name', 'STMM_segmentTemp109','StartBit', [ 16;],'SignalSize', [ 16;],'ByteOrder', 'LittleEndian','ValueType', 'SIGNED','Class', 'int16','Signed', [ 1;],'Factor', [ 0.1;],'Offset', [ 0;],'Min', [ -5;],'Max', [ 120;],'Units', 'degC','StartVal', [ 0;],'Comment', 'Segment 1 module 9','Multiplexed', [ 0;],'Multiplexor', [ 0;],'MultiplexMode_Min', [],'MultiplexMode_Max', []),struct('Name', 'STMM_segmentTemp110','StartBit', [ 32;],'SignalSize', [ 16;],'ByteOrder', 'LittleEndian','ValueType', 'SIGNED','Class', 'int16','Signed', [ 1;],'Factor', [ 0.1;],'Offset', [ 0;],'Min', [ -5;],'Max', [ 120;],'Units', 'degC','StartVal', [ 0;],'Comment', 'Segment 1 module 10','Multiplexed', [ 0;],'Multiplexor', [ 0;],'MultiplexMode_Min', [],'MultiplexMode_Max', []),struct('Name', 'STMM_segmentTemp111','StartBit', [ 48;],'SignalSize', [ 16;],'ByteOrder', 'LittleEndian','ValueType', 'SIGNED','Class', 'int16','Signed', [ 1;],'Factor', [ 0.1;],'Offset', [ 0;],'Min', [ -5;],'Max', [ 120;],'Units', 'degC','StartVal', [ 0;],'Comment', 'Segment 1 module 11','Multiplexed', [ 0;],'Multiplexor', [ 0;],'MultiplexMode_Min', [],'MultiplexMode_Max', [])}}  showRawMsg=0  useSimFunc=0  sim_func_name=''  useStartVals=0  extendedId=0
      settings: SourceProductName=Raptor
  raptor_can_rxmsg30 : Raptor_lib/CAN/raptor_can_rxmsg  canDefinition=struct('dbcFile', 'raptor_CAN2.dbc','message', 'STMM_324','comment', '','signals', {{'STMM_counterMsg324','STMM_segmentTemp700','STMM_segmentTemp701','STMM_segmentTemp702'}},'enabled', [ 1 1 1 1;],'scaled', [ 1 1 1 1;],'canBus', '''CAN2''','messageID', [ 324;],'idMask', [ 536870911;],'payloadMask', [],'payloadValue', [],'period', [ 0;],'mailbox', '''''','queueSize', [ 1;],'label', [ 1;],'ver', [ 2;],'showID', [ 0;],'showRaw', [ 0;],'showRawMsg', [ 0;],'useStartVals', [ 0;],'extendedId', [ 0;],'showAge', [ 1;],'useSimFunc', [ 0;],'sim_func_name', '''''','fill', [ 0;],'editID', [ 0;],'signalOrder', [ 1;],'signalAscDes', [ 1;],'msgLength', [ 8;])  canBus='CAN2'  mailbox=''  payloadMask=[]  payloadValue=[]  idMask=hex2dec('1FFFFFFF')  queueSize=1  showID=0  label=1  fill=0  id=324  showRaw=0  showAge=1  signalOrder=1  signalInfo={{struct('Name', 'STMM_segmentTemp702','StartBit', [ 48;],'SignalSize', [ 16;],'ByteOrder', 'LittleEndian','ValueType', 'SIGNED','Class', 'int16','Signed', [ 1;],'Factor', [ 0.1;],'Offset', [ 0;],'Min', [ -5;],'Max', [ 120;],'Units', 'degC','StartVal', [ 0;],'Comment', '','Multiplexed', [ 0;],'Multiplexor', [ 0;],'MultiplexMode_Min', [],'MultiplexMode_Max', []),struct('Name', 'STMM_segmentTemp701','StartBit', [ 32;],'SignalSize', [ 16;],'ByteOrder', 'LittleEndian','ValueType', 'SIGNED','Class', 'int16','Signed', [ 1;],'Factor', [ 0.1;],'Offset', [ 0;],'Min', [ -5;],'Max', [ 120;],'Units', 'degC','StartVal', [ 0;],'Comment', 'Segment 7 module 1','Multiplexed', [ 0;],'Multiplexor', [ 0;],'MultiplexMode_Min', [],'MultiplexMode_Max', []),struct('Name', 'STMM_segmentTemp700','StartBit', [ 16;],'SignalSize', [ 16;],'ByteOrder', 'LittleEndian','ValueType', 'SIGNED','Class', 'int16','Signed', [ 1;],'Factor', [ 0.1;],'Offset', [ 0;],'Min', [ -5;],'Max', [ 120;],'Units', 'degC','StartVal', [ 0;],'Comment', 'Segment 7 module 0','Multiplexed', [ 0;],'Multiplexor', [ 0;],'MultiplexMode_Min', [],'MultiplexMode_Max', []),struct('Name', 'STMM_counterMsg324','StartBit', [ 0;],'SignalSize', [ 4;],'ByteOrder', 'LittleEndian','ValueType', 'UNSIGNED','Class', 'uint8','Signed', [ 0;],'Factor', [ 1;],'Offset', [ 0;],'Min', [ 0;],'Max', [ 15;],'Units', '','StartVal', [ 0;],'Comment', 'Counter Message 324','Multiplexed', [ 0;],'Multiplexor', [ 0;],'MultiplexMode_Min', [],'MultiplexMode_Max', [])}}  showRawMsg=0  useSimFunc=0  sim_func_name=''  useStartVals=0  extendedId=0
      settings: SourceProductName=Raptor
  raptor_can_rxmsg31 : Raptor_lib/CAN/raptor_can_rxmsg  canDefinition=struct('dbcFile', 'raptor_CAN2.dbc','message', 'STMM_325','comment', '','signals', {{'STMM_counterMsg325','STMM_segmentTemp703','STMM_segmentTemp704','STMM_segmentTemp705'}},'enabled', [ 1 1 1 1;],'scaled', [ 1 1 1 1;],'canBus', '''CAN2''','messageID', [ 325;],'idMask', [ 536870911;],'payloadMask', [],'payloadValue', [],'period', [ 0;],'mailbox', '''''','queueSize', [ 1;],'label', [ 1;],'ver', [ 2;],'showID', [ 0;],'showRaw', [ 0;],'showRawMsg', [ 0;],'useStartVals', [ 0;],'extendedId', [ 0;],'showAge', [ 1;],'useSimFunc', [ 0;],'sim_func_name', '''''','fill', [ 0;],'editID', [ 0;],'signalOrder', [ 1;],'signalAscDes', [ 1;],'msgLength', [ 8;])  canBus='CAN2'  mailbox=''  payloadMask=[]  payloadValue=[]  idMask=hex2dec('1FFFFFFF')  queueSize=1  showID=0  label=1  fill=0  id=325  showRaw=0  showAge=1  signalOrder=1  signalInfo={{struct('Name', 'STMM_segmentTemp705','StartBit', [ 48;],'SignalSize', [ 16;],'ByteOrder', 'LittleEndian','ValueType', 'SIGNED','Class', 'int16','Signed', [ 1;],'Factor', [ 0.1;],'Offset', [ 0;],'Min', [ -5;],'Max', [ 120;],'Units', 'degC','StartVal', [ 0;],'Comment', 'Segment 7 module 5','Multiplexed', [ 0;],'Multiplexor', [ 0;],'MultiplexMode_Min', [],'MultiplexMode_Max', []),struct('Name', 'STMM_segmentTemp704','StartBit', [ 32;],'SignalSize', [ 16;],'ByteOrder', 'LittleEndian','ValueType', 'SIGNED','Class', 'int16','Signed', [ 1;],'Factor', [ 0.1;],'Offset', [ 0;],'Min', [ -5;],'Max', [ 120;],'Units', 'degC','StartVal', [ 0;],'Comment', 'Segment 7 module 4','Multiplexed', [ 0;],'Multiplexor', [ 0;],'MultiplexMode_Min', [],'MultiplexMode_Max', []),struct('Name', 'STMM_segmentTemp703','StartBit', [ 16;],'SignalSize', [ 16;],'ByteOrder', 'LittleEndian','ValueType', 'SIGNED','Class', 'int16','Signed', [ 1;],'Factor', [ 0.1;],'Offset', [ 0;],'Min', [ -5;],'Max', [ 120;],'Units', 'degC','StartVal', [ 0;],'Comment', 'Segment 7 module 3','Multiplexed', [ 0;],'Multiplexor', [ 0;],'MultiplexMode_Min', [],'MultiplexMode_Max', []),struct('Name', 'STMM_counterMsg325','StartBit', [ 0;],'SignalSize', [ 4;],'ByteOrder', 'LittleEndian','ValueType', 'UNSIGNED','Class', 'uint8','Signed', [ 0;],'Factor', [ 1;],'Offset', [ 0;],'Min', [ 0;],'Max', [ 15;],'Units', '','StartVal', [ 0;],'Comment', 'Counter Message 325','Multiplexed', [ 0;],'Multiplexor', [ 0;],'MultiplexMode_Min', [],'MultiplexMode_Max', [])}}  showRawMsg=0  useSimFunc=0  sim_func_name=''  useStartVals=0  extendedId=0
      settings: SourceProductName=Raptor
  raptor_can_rxmsg4 : Raptor_lib/CAN/raptor_can_rxmsg  canDefinition=struct('dbcFile', 'raptor_CAN2.dbc','message', 'STMM_304','comment', '','signals', {{'STMM_counterMsg304','STMM_segmentTemp200','STMM_segmentTemp201','STMM_segmentTemp202'}},'enabled', [ 1 1 1 1;],'scaled', [ 1 1 1 1;],'canBus', '''CAN2''','messageID', [ 304;],'idMask', [ 536870911;],'payloadMask', [],'payloadValue', [],'period', [ 0;],'mailbox', '''''','queueSize', [ 1;],'label', [ 1;],'ver', [ 2;],'showID', [ 0;],'showRaw', [ 0;],'showRawMsg', [ 0;],'useStartVals', [ 0;],'extendedId', [ 0;],'showAge', [ 1;],'useSimFunc', [ 0;],'sim_func_name', '''''','fill', [ 0;],'editID', [ 0;],'signalOrder', [ 1;],'signalAscDes', [ 1;],'msgLength', [ 8;])  canBus='CAN2'  mailbox=''  payloadMask=[]  payloadValue=[]  idMask=hex2dec('1FFFFFFF')  queueSize=1  showID=0  label=1  fill=0  id=304  showRaw=0  showAge=1  signalOrder=1  signalInfo={{struct('Name', 'STMM_counterMsg304','StartBit', [ 0;],'SignalSize', [ 4;],'ByteOrder', 'LittleEndian','ValueType', 'UNSIGNED','Class', 'uint8','Signed', [ 0;],'Factor', [ 1;],'Offset', [ 0;],'Min', [ 0;],'Max', [ 15;],'Units', '','StartVal', [ 0;],'Comment', 'Counter Message 304','Multiplexed', [ 0;],'Multiplexor', [ 0;],'MultiplexMode_Min', [],'MultiplexMode_Max', []),struct('Name', 'STMM_segmentTemp200','StartBit', [ 16;],'SignalSize', [ 16;],'ByteOrder', 'LittleEndian','ValueType', 'SIGNED','Class', 'int16','Signed', [ 1;],'Factor', [ 0.1;],'Offset', [ 0;],'Min', [ -5;],'Max', [ 120;],'Units', 'degC','StartVal', [ 0;],'Comment', 'Segment 2 module 0','Multiplexed', [ 0;],'Multiplexor', [ 0;],'MultiplexMode_Min', [],'MultiplexMode_Max', []),struct('Name', 'STMM_segmentTemp201','StartBit', [ 32;],'SignalSize', [ 16;],'ByteOrder', 'LittleEndian','ValueType', 'SIGNED','Class', 'int16','Signed', [ 1;],'Factor', [ 0.1;],'Offset', [ 0;],'Min', [ -5;],'Max', [ 120;],'Units', 'degC','StartVal', [ 0;],'Comment', 'Segment 2 module 1','Multiplexed', [ 0;],'Multiplexor', [ 0;],'MultiplexMode_Min', [],'MultiplexMode_Max', []),struct('Name', 'STMM_segmentTemp202','StartBit', [ 48;],'SignalSize', [ 16;],'ByteOrder', 'LittleEndian','ValueType', 'SIGNED','Class', 'int16','Signed', [ 1;],'Factor', [ 0.1;],'Offset', [ 0;],'Min', [ -5;],'Max', [ 120;],'Units', 'degC','StartVal', [ 0;],'Comment', 'Segment 2 module 2','Multiplexed', [ 0;],'Multiplexor', [ 0;],'MultiplexMode_Min', [],'MultiplexMode_Max', [])}}  showRawMsg=0  useSimFunc=0  sim_func_name=''  useStartVals=0  extendedId=0
      settings: SourceProductName=Raptor
  raptor_can_rxmsg5 : Raptor_lib/CAN/raptor_can_rxmsg  canDefinition=struct('dbcFile', 'raptor_CAN2.dbc','message', 'STMM_305','comment', '','signals', {{'STMM_counterMsg305','STMM_segmentTemp203','STMM_segmentTemp204','STMM_segmentTemp205'}},'enabled', [ 1 1 1 1;],'scaled', [ 1 1 1 1;],'canBus', '''CAN2''','messageID', [ 305;],'idMask', [ 536870911;],'payloadMask', [],'payloadValue', [],'period', [ 0;],'mailbox', '''''','queueSize', [ 1;],'label', [ 1;],'ver', [ 2;],'showID', [ 0;],'showRaw', [ 0;],'showRawMsg', [ 0;],'useStartVals', [ 0;],'extendedId', [ 0;],'showAge', [ 1;],'useSimFunc', [ 0;],'sim_func_name', '''''','fill', [ 0;],'editID', [ 0;],'signalOrder', [ 1;],'signalAscDes', [ 1;],'msgLength', [ 8;])  canBus='CAN2'  mailbox=''  payloadMask=[]  payloadValue=[]  idMask=hex2dec('1FFFFFFF')  queueSize=1  showID=0  label=1  fill=0  id=305  showRaw=0  showAge=1  signalOrder=1  signalInfo={{struct('Name', 'STMM_counterMsg305','StartBit', [ 0;],'SignalSize', [ 4;],'ByteOrder', 'LittleEndian','ValueType', 'UNSIGNED','Class', 'uint8','Signed', [ 0;],'Factor', [ 1;],'Offset', [ 0;],'Min', [ 0;],'Max', [ 15;],'Units', '','StartVal', [ 0;],'Comment', 'Counter Message 305','Multiplexed', [ 0;],'Multiplexor', [ 0;],'MultiplexMode_Min', [],'MultiplexMode_Max', []),struct('Name', 'STMM_segmentTemp203','StartBit', [ 16;],'SignalSize', [ 16;],'ByteOrder', 'LittleEndian','ValueType', 'SIGNED','Class', 'int16','Signed', [ 1;],'Factor', [ 0.1;],'Offset', [ 0;],'Min', [ -5;],'Max', [ 120;],'Units', 'degC','StartVal', [ 0;],'Comment', 'Segment 2 module 3','Multiplexed', [ 0;],'Multiplexor', [ 0;],'MultiplexMode_Min', [],'MultiplexMode_Max', []),struct('Name', 'STMM_segmentTemp204','StartBit', [ 32;],'SignalSize', [ 16;],'ByteOrder', 'LittleEndian','ValueType', 'SIGNED','Class', 'int16','Signed', [ 1;],'Factor', [ 0.1;],'Offset', [ 0;],'Min', [ -5;],'Max', [ 120;],'Units', 'degC','StartVal', [ 0;],'Comment', 'Segment 2 module 4','Multiplexed', [ 0;],'Multiplexor', [ 0;],'MultiplexMode_Min', [],'MultiplexMode_Max', []),struct('Name', 'STMM_segmentTemp205','StartBit', [ 48;],'SignalSize', [ 16;],'ByteOrder', 'LittleEndian','ValueType', 'SIGNED','Class', 'int16','Signed', [ 1;],'Factor', [ 0.1;],'Offset', [ 0;],'Min', [ -5;],'Max', [ 120;],'Units', 'degC','StartVal', [ 0;],'Comment', 'Segment 2 module 5','Multiplexed', [ 0;],'Multiplexor', [ 0;],'MultiplexMode_Min', [],'MultiplexMode_Max', [])}}  showRawMsg=0  useSimFunc=0  sim_func_name=''  useStartVals=0  extendedId=0
      settings: SourceProductName=Raptor
  raptor_can_rxmsg6 : Raptor_lib/CAN/raptor_can_rxmsg  canDefinition=struct('dbcFile', 'raptor_CAN2.dbc','message', 'STMM_306','comment', '','signals', {{'STMM_counterMsg306','STMM_segmentTemp206','STMM_segmentTemp207','STMM_segmentTemp208'}},'enabled', [ 1 1 1 1;],'scaled', [ 1 1 1 1;],'canBus', '''CAN2''','messageID', [ 306;],'idMask', [ 536870911;],'payloadMask', [],'payloadValue', [],'period', [ 0;],'mailbox', '''''','queueSize', [ 1;],'label', [ 1;],'ver', [ 2;],'showID', [ 0;],'showRaw', [ 0;],'showRawMsg', [ 0;],'useStartVals', [ 0;],'extendedId', [ 0;],'showAge', [ 1;],'useSimFunc', [ 0;],'sim_func_name', '''''','fill', [ 0;],'editID', [ 0;],'signalOrder', [ 1;],'signalAscDes', [ 1;],'msgLength', [ 8;])  canBus='CAN2'  mailbox=''  payloadMask=[]  payloadValue=[]  idMask=hex2dec('1FFFFFFF')  queueSize=1  showID=0  label=1  fill=0  id=306  showRaw=0  showAge=1  signalOrder=1  signalInfo={{struct('Name', 'STMM_counterMsg306','StartBit', [ 0;],'SignalSize', [ 4;],'ByteOrder', 'LittleEndian','ValueType', 'UNSIGNED','Class', 'uint8','Signed', [ 0;],'Factor', [ 1;],'Offset', [ 0;],'Min', [ 0;],'Max', [ 15;],'Units', '','StartVal', [ 0;],'Comment', 'Counter Message 306','Multiplexed', [ 0;],'Multiplexor', [ 0;],'MultiplexMode_Min', [],'MultiplexMode_Max', []),struct('Name', 'STMM_segmentTemp206','StartBit', [ 16;],'SignalSize', [ 16;],'ByteOrder', 'LittleEndian','ValueType', 'SIGNED','Class', 'int16','Signed', [ 1;],'Factor', [ 0.1;],'Offset', [ 0;],'Min', [ -5;],'Max', [ 120;],'Units', 'degC','StartVal', [ 0;],'Comment', 'Segment 2 module 6','Multiplexed', [ 0;],'Multiplexor', [ 0;],'MultiplexMode_Min', [],'MultiplexMode_Max', []),struct('Name', 'STMM_segmentTemp207','StartBit', [ 32;],'SignalSize', [ 16;],'ByteOrder', 'LittleEndian','ValueType', 'SIGNED','Class', 'int16','Signed', [ 1;],'Factor', [ 0.1;],'Offset', [ 0;],'Min', [ -5;],'Max', [ 120;],'Units', 'degC','StartVal', [ 0;],'Comment', 'Segment 2 module 7','Multiplexed', [ 0;],'Multiplexor', [ 0;],'MultiplexMode_Min', [],'MultiplexMode_Max', []),struct('Name', 'STMM_segmentTemp208','StartBit', [ 48;],'SignalSize', [ 16;],'ByteOrder', 'LittleEndian','ValueType', 'SIGNED','Class', 'int16','Signed', [ 1;],'Factor', [ 0.1;],'Offset', [ 0;],'Min', [ -5;],'Max', [ 120;],'Units', 'degC','StartVal', [ 0;],'Comment', 'Segment 2 module 8','Multiplexed', [ 0;],'Multiplexor', [ 0;],'MultiplexMode_Min', [],'MultiplexMode_Max', [])}}  showRawMsg=0  useSimFunc=0  sim_func_name=''  useStartVals=0  extendedId=0
      settings: SourceProductName=Raptor
  raptor_can_rxmsg7 : Raptor_lib/CAN/raptor_can_rxmsg  canDefinition=struct('dbcFile', 'raptor_CAN2.dbc','message', 'STMM_307','comment', '','signals', {{'STMM_counterMsg307','STMM_segmentTemp209','STMM_segmentTemp210','STMM_segmentTemp211'}},'enabled', [ 1 1 1 1;],'scaled', [ 1 1 1 1;],'canBus', '''CAN2''','messageID', [ 307;],'idMask', [ 536870911;],'payloadMask', [],'payloadValue', [],'period', [ 0;],'mailbox', '''''','queueSize', [ 1;],'label', [ 1;],'ver', [ 2;],'showID', [ 0;],'showRaw', [ 0;],'showRawMsg', [ 0;],'useStartVals', [ 0;],'extendedId', [ 0;],'showAge', [ 1;],'useSimFunc', [ 0;],'sim_func_name', '''''','fill', [ 0;],'editID', [ 0;],'signalOrder', [ 1;],'signalAscDes', [ 1;],'msgLength', [ 8;])  canBus='CAN2'  mailbox=''  payloadMask=[]  payloadValue=[]  idMask=hex2dec('1FFFFFFF')  queueSize=1  showID=0  label=1  fill=0  id=307  showRaw=0  showAge=1  signalOrder=1  signalInfo={{struct('Name', 'STMM_counterMsg307','StartBit', [ 0;],'SignalSize', [ 4;],'ByteOrder', 'LittleEndian','ValueType', 'UNSIGNED','Class', 'uint8','Signed', [ 0;],'Factor', [ 1;],'Offset', [ 0;],'Min', [ 0;],'Max', [ 15;],'Units', '','StartVal', [ 0;],'Comment', 'Counter Message 307','Multiplexed', [ 0;],'Multiplexor', [ 0;],'MultiplexMode_Min', [],'MultiplexMode_Max', []),struct('Name', 'STMM_segmentTemp209','StartBit', [ 16;],'SignalSize', [ 16;],'ByteOrder', 'LittleEndian','ValueType', 'SIGNED','Class', 'int16','Signed', [ 1;],'Factor', [ 0.1;],'Offset', [ 0;],'Min', [ -5;],'Max', [ 120;],'Units', 'degC','StartVal', [ 0;],'Comment', 'Segment 2 module 9','Multiplexed', [ 0;],'Multiplexor', [ 0;],'MultiplexMode_Min', [],'MultiplexMode_Max', []),struct('Name', 'STMM_segmentTemp210','StartBit', [ 32;],'SignalSize', [ 16;],'ByteOrder', 'LittleEndian','ValueType', 'SIGNED','Class', 'int16','Signed', [ 1;],'Factor', [ 0.1;],'Offset', [ 0;],'Min', [ -5;],'Max', [ 120;],'Units', 'degC','StartVal', [ 0;],'Comment', 'Segment 2 module 10','Multiplexed', [ 0;],'Multiplexor', [ 0;],'MultiplexMode_Min', [],'MultiplexMode_Max', []),struct('Name', 'STMM_segmentTemp211','StartBit', [ 48;],'SignalSize', [ 16;],'ByteOrder', 'LittleEndian','ValueType', 'SIGNED','Class', 'int16','Signed', [ 1;],'Factor', [ 0.1;],'Offset', [ 0;],'Min', [ -5;],'Max', [ 120;],'Units', 'degC','StartVal', [ 0;],'Comment', 'Segment 2 module 11','Multiplexed', [ 0;],'Multiplexor', [ 0;],'MultiplexMode_Min', [],'MultiplexMode_Max', [])}}  showRawMsg=0  useSimFunc=0  sim_func_name=''  useStartVals=0  extendedId=0
      settings: SourceProductName=Raptor
  raptor_can_rxmsg8 : Raptor_lib/CAN/raptor_can_rxmsg  canDefinition=struct('dbcFile', 'raptor_CAN2.dbc','message', 'STMM_308','comment', '','signals', {{'STMM_counterMsg308','STMM_segmentTemp300','STMM_segmentTemp301','STMM_segmentTemp302'}},'enabled', [ 1 1 1 1;],'scaled', [ 1 1 1 1;],'canBus', '''CAN2''','messageID', [ 308;],'idMask', [ 536870911;],'payloadMask', [],'payloadValue', [],'period', [ 0;],'mailbox', '''''','queueSize', [ 1;],'label', [ 1;],'ver', [ 2;],'showID', [ 0;],'showRaw', [ 0;],'showRawMsg', [ 0;],'useStartVals', [ 0;],'extendedId', [ 0;],'showAge', [ 1;],'useSimFunc', [ 0;],'sim_func_name', '''''','fill', [ 0;],'editID', [ 0;],'signalOrder', [ 1;],'signalAscDes', [ 1;],'msgLength', [ 8;])  canBus='CAN2'  mailbox=''  payloadMask=[]  payloadValue=[]  idMask=hex2dec('1FFFFFFF')  queueSize=1  showID=0  label=1  fill=0  id=308  showRaw=0  showAge=1  signalOrder=1  signalInfo={{struct('Name', 'STMM_counterMsg308','StartBit', [ 0;],'SignalSize', [ 4;],'ByteOrder', 'LittleEndian','ValueType', 'UNSIGNED','Class', 'uint8','Signed', [ 0;],'Factor', [ 1;],'Offset', [ 0;],'Min', [ 0;],'Max', [ 15;],'Units', '','StartVal', [ 0;],'Comment', 'Counter Message 308','Multiplexed', [ 0;],'Multiplexor', [ 0;],'MultiplexMode_Min', [],'MultiplexMode_Max', []),struct('Name', 'STMM_segmentTemp300','StartBit', [ 16;],'SignalSize', [ 16;],'ByteOrder', 'LittleEndian','ValueType', 'SIGNED','Class', 'int16','Signed', [ 1;],'Factor', [ 0.1;],'Offset', [ 0;],'Min', [ -5;],'Max', [ 120;],'Units', 'degC','StartVal', [ 0;],'Comment', 'Segment 3 module 0','Multiplexed', [ 0;],'Multiplexor', [ 0;],'MultiplexMode_Min', [],'MultiplexMode_Max', []),struct('Name', 'STMM_segmentTemp301','StartBit', [ 32;],'SignalSize', [ 16;],'ByteOrder', 'LittleEndian','ValueType', 'SIGNED','Class', 'int16','Signed', [ 1;],'Factor', [ 0.1;],'Offset', [ 0;],'Min', [ -5;],'Max', [ 120;],'Units', 'degC','StartVal', [ 0;],'Comment', 'Segment 3 module 1','Multiplexed', [ 0;],'Multiplexor', [ 0;],'MultiplexMode_Min', [],'MultiplexMode_Max', []),struct('Name', 'STMM_segmentTemp302','StartBit', [ 48;],'SignalSize', [ 16;],'ByteOrder', 'LittleEndian','ValueType', 'SIGNED','Class', 'int16','Signed', [ 1;],'Factor', [ 0.1;],'Offset', [ 0;],'Min', [ -5;],'Max', [ 120;],'Units', 'degC','StartVal', [ 0;],'Comment', 'Segment 3 module 2','Multiplexed', [ 0;],'Multiplexor', [ 0;],'MultiplexMode_Min', [],'MultiplexMode_Max', [])}}  showRawMsg=0  useSimFunc=0  sim_func_name=''  useStartVals=0  extendedId=0
      settings: SourceProductName=Raptor
  raptor_can_rxmsg9 : Raptor_lib/CAN/raptor_can_rxmsg  canDefinition=struct('dbcFile', 'raptor_CAN2.dbc','message', 'STMM_309','comment', '','signals', {{'STMM_counterMsg309','STMM_segmentTemp303','STMM_segmentTemp304','STMM_segmentTemp305'}},'enabled', [ 1 1 1 1;],'scaled', [ 1 1 1 1;],'canBus', '''CAN2''','messageID', [ 309;],'idMask', [ 536870911;],'payloadMask', [],'payloadValue', [],'period', [ 0;],'mailbox', '''''','queueSize', [ 1;],'label', [ 1;],'ver', [ 2;],'showID', [ 0;],'showRaw', [ 0;],'showRawMsg', [ 0;],'useStartVals', [ 0;],'extendedId', [ 0;],'showAge', [ 1;],'useSimFunc', [ 0;],'sim_func_name', '''''','fill', [ 0;],'editID', [ 0;],'signalOrder', [ 1;],'signalAscDes', [ 1;],'msgLength', [ 8;])  canBus='CAN2'  mailbox=''  payloadMask=[]  payloadValue=[]  idMask=hex2dec('1FFFFFFF')  queueSize=1  showID=0  label=1  fill=0  id=309  showRaw=0  showAge=1  signalOrder=1  signalInfo={{struct('Name', 'STMM_counterMsg309','StartBit', [ 0;],'SignalSize', [ 4;],'ByteOrder', 'LittleEndian','ValueType', 'UNSIGNED','Class', 'uint8','Signed', [ 0;],'Factor', [ 1;],'Offset', [ 0;],'Min', [ 0;],'Max', [ 15;],'Units', '','StartVal', [ 0;],'Comment', 'Counter Message 309','Multiplexed', [ 0;],'Multiplexor', [ 0;],'MultiplexMode_Min', [],'MultiplexMode_Max', []),struct('Name', 'STMM_segmentTemp303','StartBit', [ 16;],'SignalSize', [ 16;],'ByteOrder', 'LittleEndian','ValueType', 'SIGNED','Class', 'int16','Signed', [ 1;],'Factor', [ 0.1;],'Offset', [ 0;],'Min', [ -5;],'Max', [ 120;],'Units', 'degC','StartVal', [ 0;],'Comment', 'Segment 3 module 3','Multiplexed', [ 0;],'Multiplexor', [ 0;],'MultiplexMode_Min', [],'MultiplexMode_Max', []),struct('Name', 'STMM_segmentTemp304','StartBit', [ 32;],'SignalSize', [ 16;],'ByteOrder', 'LittleEndian','ValueType', 'SIGNED','Class', 'int16','Signed', [ 1;],'Factor', [ 0.1;],'Offset', [ 0;],'Min', [ -5;],'Max', [ 120;],'Units', 'degC','StartVal', [ 0;],'Comment', 'Segment 3 module 4','Multiplexed', [ 0;],'Multiplexor', [ 0;],'MultiplexMode_Min', [],'MultiplexMode_Max', []),struct('Name', 'STMM_segmentTemp305','StartBit', [ 48;],'SignalSize', [ 16;],'ByteOrder', 'LittleEndian','ValueType', 'SIGNED','Class', 'int16','Signed', [ 1;],'Factor', [ 0.1;],'Offset', [ 0;],'Min', [ -5;],'Max', [ 120;],'Units', 'degC','StartVal', [ 0;],'Comment', 'Segment 3 module 5','Multiplexed', [ 0;],'Multiplexor', [ 0;],'MultiplexMode_Min', [],'MultiplexMode_Max', [])}}  showRawMsg=0  useSimFunc=0  sim_func_name=''  useStartVals=0  extendedId=0
      settings: SourceProductName=Raptor
  IO_CAN2_STMM_Bus : Outport
  wires:
  Bus Creator32/1 -> IO_CAN2_STMM_Bus/1  "IO_CAN2_STMM_Bus"
  [IO_CAN2_331_Bus] -> Bus Creator32/32
  [IO_CAN2_330_Bus] -> Bus Creator32/31
  [IO_CAN2_329_Bus] -> Bus Creator32/30
  [IO_CAN2_328_Bus] -> Bus Creator32/29
  [IO_CAN2_327_Bus] -> Bus Creator32/28
  [IO_CAN2_326_Bus] -> Bus Creator32/27
  [IO_CAN2_325_Bus] -> Bus Creator32/26
  [IO_CAN2_324_Bus] -> Bus Creator32/25
  [IO_CAN2_323_Bus] -> Bus Creator32/24
  [IO_CAN2_322_Bus] -> Bus Creator32/23
  [IO_CAN2_321_Bus] -> Bus Creator32/22
  [IO_CAN2_320_Bus] -> Bus Creator32/21
  [IO_CAN2_319_Bus] -> Bus Creator32/20
  [IO_CAN2_318_Bus] -> Bus Creator32/19
  [IO_CAN2_317_Bus] -> Bus Creator32/18
  [IO_CAN2_316_Bus] -> Bus Creator32/17
  [IO_CAN2_315_Bus] -> Bus Creator32/16
  [IO_CAN2_314_Bus] -> Bus Creator32/15
  [IO_CAN2_313_Bus] -> Bus Creator32/14
  [IO_CAN2_312_Bus] -> Bus Creator32/13
  [IO_CAN2_311_Bus] -> Bus Creator32/12
  [IO_CAN2_310_Bus] -> Bus Creator32/11
  [IO_CAN2_309_Bus] -> Bus Creator32/10
  [IO_CAN2_308_Bus] -> Bus Creator32/9
  [IO_CAN2_307_Bus] -> Bus Creator32/8
  [IO_CAN2_306_Bus] -> Bus Creator32/7
  [IO_CAN2_305_Bus] -> Bus Creator32/6
  [IO_CAN2_304_Bus] -> Bus Creator32/5
  [IO_CAN2_303_Bus] -> Bus Creator32/4
  [IO_CAN2_302_Bus] -> Bus Creator32/3
  [IO_CAN2_301_Bus] -> Bus Creator32/2
  [IO_CAN2_300_Bus] -> Bus Creator32/1
  Bus Creator27/1 -> [IO_CAN2_331_Bus]  "IO_CAN2_331_Bus"
  Bus Creator26/1 -> [IO_CAN2_330_Bus]  "IO_CAN2_330_Bus"
  Bus Creator29/1 -> [IO_CAN2_329_Bus]  "IO_CAN2_329_Bus"
  Bus Creator28/1 -> [IO_CAN2_328_Bus]  "IO_CAN2_328_Bus"
  Bus Creator25/1 -> [IO_CAN2_327_Bus]  "IO_CAN2_327_Bus"
  Bus Creator24/1 -> [IO_CAN2_326_Bus]  "IO_CAN2_326_Bus"
  Bus Creator31/1 -> [IO_CAN2_325_Bus]  "IO_CAN2_325_Bus"
  Bus Creator30/1 -> [IO_CAN2_324_Bus]  "IO_CAN2_324_Bus"
  Bus Creator19/1 -> [IO_CAN2_323_Bus]  "IO_CAN2_323_Bus"
  Bus Creator18/1 -> [IO_CAN2_322_Bus]  "IO_CAN2_322_Bus"
  Bus Creator21/1 -> [IO_CAN2_321_Bus]  "IO_CAN2_321_Bus"
  Bus Creator20/1 -> [IO_CAN2_320_Bus]  "IO_CAN2_320_Bus"
  Bus Creator17/1 -> [IO_CAN2_319_Bus]  "IO_CAN2_319_Bus"
  Bus Creator16/1 -> [IO_CAN2_318_Bus]  "IO_CAN2_318_Bus"
  Bus Creator23/1 -> [IO_CAN2_317_Bus]  "IO_CAN2_317_Bus"
  Bus Creator22/1 -> [IO_CAN2_316_Bus]  "IO_CAN2_316_Bus"
  Bus Creator13/1 -> [IO_CAN2_315_Bus]  "IO_CAN2_315_Bus"
  Bus Creator12/1 -> [IO_CAN2_314_Bus]  "IO_CAN2_314_Bus"
  Bus Creator15/1 -> [IO_CAN2_313_Bus]  "IO_CAN2_313_Bus"
  Bus Creator14/1 -> [IO_CAN2_312_Bus]  "IO_CAN2_312_Bus"
  Bus Creator11/1 -> [IO_CAN2_311_Bus]  "IO_CAN2_311_Bus"
  Bus Creator10/1 -> [IO_CAN2_310_Bus]  "IO_CAN2_310_Bus"
  Bus Creator9/1 -> [IO_CAN2_309_Bus]  "IO_CAN2_309_Bus"
  Bus Creator8/1 -> [IO_CAN2_308_Bus]  "IO_CAN2_308_Bus"
  Bus Creator7/1 -> [IO_CAN2_307_Bus]  "IO_CAN2_307_Bus"
  Bus Creator6/1 -> [IO_CAN2_306_Bus]  "IO_CAN2_306_Bus"
  Bus Creator5/1 -> [IO_CAN2_305_Bus]  "IO_CAN2_305_Bus"
  Bus Creator4/1 -> [IO_CAN2_304_Bus]  "IO_CAN2_304_Bus"
  Bus Creator3/1 -> [IO_CAN2_303_Bus]  "IO_CAN2_303_Bus"
  Bus Creator2/1 -> [IO_CAN2_302_Bus]  "IO_CAN2_302_Bus"
  Bus Creator1/1 -> [IO_CAN2_301_Bus]  "IO_CAN2_301_Bus"
  Bus Creator/1 -> [IO_CAN2_300_Bus]  "IO_CAN2_300_Bus"
  raptor_can_rxmsg29/2 -> Bus Creator29/2  "STMM_counterMsg329"
  raptor_can_rxmsg28/5 -> Bus Creator28/5  "STMM_segmentTemp802"
  raptor_can_rxmsg28/4 -> Bus Creator28/4  "STMM_segmentTemp801"
  raptor_can_rxmsg27/1 -> Bus Creator27/1  "Age"
  raptor_can_rxmsg27/2 -> Bus Creator27/2  "STMM_counterMsg331"
  raptor_can_rxmsg29/3 -> Bus Creator29/3  "STMM_segmentTemp803"
  raptor_can_rxmsg28/2 -> Bus Creator28/2  "STMM_counterMsg328"
  raptor_can_rxmsg29/1 -> Bus Creator29/1  "Age"
  raptor_can_rxmsg29/5 -> Bus Creator29/5  "STMM_segmentTemp805"
  raptor_can_rxmsg27/4 -> Bus Creator27/4  "STMM_segmentTemp810"
  raptor_can_rxmsg25/5 -> Bus Creator25/5  "STMM_segmentTemp711"
  raptor_can_rxmsg26/3 -> Bus Creator26/3  "STMM_segmentTemp806"
  raptor_can_rxmsg30/3 -> Bus Creator30/3  "STMM_segmentTemp700"
  raptor_can_rxmsg27/5 -> Bus Creator27/5  "STMM_segmentTemp811"
  raptor_can_rxmsg27/3 -> Bus Creator27/3  "STMM_segmentTemp809"
  raptor_can_rxmsg25/2 -> Bus Creator25/2  "STMM_counterMsg327"
  raptor_can_rxmsg28/1 -> Bus Creator28/1  "Age"
  raptor_can_rxmsg29/4 -> Bus Creator29/4  "STMM_segmentTemp804"
  raptor_can_rxmsg24/5 -> Bus Creator24/5  "STMM_segmentTemp708"
  raptor_can_rxmsg30/4 -> Bus Creator30/4  "STMM_segmentTemp701"
  raptor_can_rxmsg25/1 -> Bus Creator25/1  "Age"
  raptor_can_rxmsg24/2 -> Bus Creator24/2  "STMM_counterMsg326"
  raptor_can_rxmsg26/1 -> Bus Creator26/1  "Age"
  raptor_can_rxmsg31/2 -> Bus Creator31/2  "STMM_counterMsg325"
  raptor_can_rxmsg26/4 -> Bus Creator26/4  "STMM_segmentTemp807"
  raptor_can_rxmsg30/1 -> Bus Creator30/1  "Age"
  raptor_can_rxmsg26/5 -> Bus Creator26/5  "STMM_segmentTemp808"
  raptor_can_rxmsg24/3 -> Bus Creator24/3  "STMM_segmentTemp706"
  raptor_can_rxmsg28/3 -> Bus Creator28/3  "STMM_segmentTemp800"
  raptor_can_rxmsg25/3 -> Bus Creator25/3  "STMM_segmentTemp709"
  raptor_can_rxmsg24/1 -> Bus Creator24/1  "Age"
  raptor_can_rxmsg31/5 -> Bus Creator31/5  "STMM_segmentTemp705"
  raptor_can_rxmsg30/5 -> Bus Creator30/5  "STMM_segmentTemp702"
  raptor_can_rxmsg24/4 -> Bus Creator24/4  "STMM_segmentTemp707"
  raptor_can_rxmsg25/4 -> Bus Creator25/4  "STMM_segmentTemp710"
  raptor_can_rxmsg30/2 -> Bus Creator30/2  "STMM_counterMsg324"
  raptor_can_rxmsg31/1 -> Bus Creator31/1  "Age"
  raptor_can_rxmsg31/3 -> Bus Creator31/3  "STMM_segmentTemp703"
  raptor_can_rxmsg31/4 -> Bus Creator31/4  "STMM_segmentTemp704"
  raptor_can_rxmsg26/2 -> Bus Creator26/2  "STMM_counterMsg330"
  raptor_can_rxmsg23/4 -> Bus Creator23/4  "STMM_segmentTemp504"
  raptor_can_rxmsg23/3 -> Bus Creator23/3  "STMM_segmentTemp503"
  raptor_can_rxmsg20/1 -> Bus Creator20/1  "Age"
  raptor_can_rxmsg18/2 -> Bus Creator18/2  "STMM_counterMsg322"
  raptor_can_rxmsg17/3 -> Bus Creator17/3  "STMM_segmentTemp509"
  raptor_can_rxmsg19/2 -> Bus Creator19/2  "STMM_counterMsg323"
  raptor_can_rxmsg17/4 -> Bus Creator17/4  "STMM_segmentTemp510"
  raptor_can_rxmsg20/4 -> Bus Creator20/4  "STMM_segmentTemp601"
  raptor_can_rxmsg22/2 -> Bus Creator22/2  "STMM_counterMsg316"
  raptor_can_rxmsg23/1 -> Bus Creator23/1  "Age"
  raptor_can_rxmsg16/4 -> Bus Creator16/4  "STMM_segmentTemp507"
  raptor_can_rxmsg23/5 -> Bus Creator23/5  "STMM_segmentTemp505"
  raptor_can_rxmsg16/3 -> Bus Creator16/3  "STMM_segmentTemp506"
  raptor_can_rxmsg18/5 -> Bus Creator18/5  "STMM_segmentTemp608"
  raptor_can_rxmsg20/3 -> Bus Creator20/3  "STMM_segmentTemp600"
  raptor_can_rxmsg22/5 -> Bus Creator22/5  "STMM_segmentTemp502"
  raptor_can_rxmsg16/2 -> Bus Creator16/2  "STMM_counterMsg318"
  raptor_can_rxmsg22/3 -> Bus Creator22/3  "STMM_segmentTemp500"
  raptor_can_rxmsg16/1 -> Bus Creator16/1  "Age"
  raptor_can_rxmsg22/1 -> Bus Creator22/1  "Age"
  raptor_can_rxmsg23/2 -> Bus Creator23/2  "STMM_counterMsg317"
  raptor_can_rxmsg17/5 -> Bus Creator17/5  "STMM_segmentTemp511"
  raptor_can_rxmsg18/1 -> Bus Creator18/1  "Age"
  raptor_can_rxmsg17/1 -> Bus Creator17/1  "Age"
  raptor_can_rxmsg16/5 -> Bus Creator16/5  "STMM_segmentTemp508"
  raptor_can_rxmsg17/2 -> Bus Creator17/2  "STMM_counterMsg319"
  raptor_can_rxmsg21/4 -> Bus Creator21/4  "STMM_segmentTemp604"
  raptor_can_rxmsg22/4 -> Bus Creator22/4  "STMM_segmentTemp501"
  raptor_can_rxmsg18/4 -> Bus Creator18/4  "STMM_segmentTemp607"
  raptor_can_rxmsg20/5 -> Bus Creator20/5  "STMM_segmentTemp602"
  raptor_can_rxmsg19/3 -> Bus Creator19/3  "STMM_segmentTemp609"
  raptor_can_rxmsg21/5 -> Bus Creator21/5  "STMM_segmentTemp605"
  raptor_can_rxmsg20/2 -> Bus Creator20/2  "STMM_counterMsg320"
  raptor_can_rxmsg18/3 -> Bus Creator18/3  "STMM_segmentTemp606"
  raptor_can_rxmsg21/3 -> Bus Creator21/3  "STMM_segmentTemp603"
  raptor_can_rxmsg21/2 -> Bus Creator21/2  "STMM_counterMsg321"
  raptor_can_rxmsg19/5 -> Bus Creator19/5  "STMM_segmentTemp611"
  raptor_can_rxmsg19/4 -> Bus Creator19/4  "STMM_segmentTemp610"
  raptor_can_rxmsg19/1 -> Bus Creator19/1  "Age"
  raptor_can_rxmsg21/1 -> Bus Creator21/1  "Age"
  raptor_can_rxmsg15/4 -> Bus Creator15/4  "STMM_segmentTemp404"
  raptor_can_rxmsg15/3 -> Bus Creator15/3  "STMM_segmentTemp403"
  raptor_can_rxmsg12/3 -> Bus Creator12/3  "STMM_segmentTemp406"
  raptor_can_rxmsg14/2 -> Bus Creator14/2  "STMM_counterMsg312"
  raptor_can_rxmsg15/1 -> Bus Creator15/1  "Age"
  raptor_can_rxmsg12/4 -> Bus Creator12/4  "STMM_segmentTemp407"
  raptor_can_rxmsg15/5 -> Bus Creator15/5  "STMM_segmentTemp405"
  raptor_can_rxmsg13/3 -> Bus Creator13/3  "STMM_segmentTemp409"
  raptor_can_rxmsg14/5 -> Bus Creator14/5  "STMM_segmentTemp402"
  raptor_can_rxmsg12/2 -> Bus Creator12/2  "STMM_counterMsg314"
  raptor_can_rxmsg14/3 -> Bus Creator14/3  "STMM_segmentTemp400"
  raptor_can_rxmsg12/1 -> Bus Creator12/1  "Age"
  raptor_can_rxmsg14/1 -> Bus Creator14/1  "Age"
  raptor_can_rxmsg13/4 -> Bus Creator13/4  "STMM_segmentTemp410"
  raptor_can_rxmsg15/2 -> Bus Creator15/2  "STMM_counterMsg313"
  raptor_can_rxmsg13/5 -> Bus Creator13/5  "STMM_segmentTemp411"
  raptor_can_rxmsg13/1 -> Bus Creator13/1  "Age"
  raptor_can_rxmsg12/5 -> Bus Creator12/5  "STMM_segmentTemp408"
  raptor_can_rxmsg13/2 -> Bus Creator13/2  "STMM_counterMsg315"
  raptor_can_rxmsg14/4 -> Bus Creator14/4  "STMM_segmentTemp401"
  raptor_can_rxmsg11/2 -> Bus Creator11/2  "STMM_counterMsg311"
  raptor_can_rxmsg8/4 -> Bus Creator8/4  "STMM_segmentTemp301"
  raptor_can_rxmsg11/5 -> Bus Creator11/5  "STMM_segmentTemp311"
  raptor_can_rxmsg11/4 -> Bus Creator11/4  "STMM_segmentTemp310"
  raptor_can_rxmsg10/5 -> Bus Creator10/5  "STMM_segmentTemp308"
  raptor_can_rxmsg9/2 -> Bus Creator9/2  "STMM_counterMsg309"
  raptor_can_rxmsg11/1 -> Bus Creator11/1  "Age"
  raptor_can_rxmsg8/5 -> Bus Creator8/5  "STMM_segmentTemp302"
  raptor_can_rxmsg10/2 -> Bus Creator10/2  "STMM_counterMsg310"
  raptor_can_rxmsg10/3 -> Bus Creator10/3  "STMM_segmentTemp306"
  raptor_can_rxmsg8/1 -> Bus Creator8/1  "Age"
  raptor_can_rxmsg8/3 -> Bus Creator8/3  "STMM_segmentTemp300"
  raptor_can_rxmsg10/1 -> Bus Creator10/1  "Age"
  raptor_can_rxmsg9/5 -> Bus Creator9/5  "STMM_segmentTemp305"
  raptor_can_rxmsg11/3 -> Bus Creator11/3  "STMM_segmentTemp309"
  raptor_can_rxmsg10/4 -> Bus Creator10/4  "STMM_segmentTemp307"
  raptor_can_rxmsg8/2 -> Bus Creator8/2  "STMM_counterMsg308"
  raptor_can_rxmsg9/3 -> Bus Creator9/3  "STMM_segmentTemp303"
  raptor_can_rxmsg9/1 -> Bus Creator9/1  "Age"
  raptor_can_rxmsg9/4 -> Bus Creator9/4  "STMM_segmentTemp304"
  raptor_can_rxmsg7/5 -> Bus Creator7/5  "STMM_segmentTemp211"
  raptor_can_rxmsg7/4 -> Bus Creator7/4  "STMM_segmentTemp210"
  raptor_can_rxmsg7/3 -> Bus Creator7/3  "STMM_segmentTemp209"
  raptor_can_rxmsg7/2 -> Bus Creator7/2  "STMM_counterMsg307"
  raptor_can_rxmsg7/1 -> Bus Creator7/1  "Age"
  raptor_can_rxmsg6/5 -> Bus Creator6/5  "STMM_segmentTemp208"
  raptor_can_rxmsg6/4 -> Bus Creator6/4  "STMM_segmentTemp207"
  raptor_can_rxmsg6/3 -> Bus Creator6/3  "STMM_segmentTemp206"
  raptor_can_rxmsg6/2 -> Bus Creator6/2  "STMM_counterMsg306"
  raptor_can_rxmsg6/1 -> Bus Creator6/1  "Age"
  raptor_can_rxmsg5/5 -> Bus Creator5/5  "STMM_segmentTemp205"
  raptor_can_rxmsg5/4 -> Bus Creator5/4  "STMM_segmentTemp204"
  raptor_can_rxmsg5/3 -> Bus Creator5/3  "STMM_segmentTemp203"
  raptor_can_rxmsg5/2 -> Bus Creator5/2  "STMM_counterMsg305"
  raptor_can_rxmsg5/1 -> Bus Creator5/1  "Age"
  raptor_can_rxmsg4/5 -> Bus Creator4/5  "STMM_segmentTemp202"
  raptor_can_rxmsg4/4 -> Bus Creator4/4  "STMM_segmentTemp201"
  raptor_can_rxmsg4/3 -> Bus Creator4/3  "STMM_segmentTemp200"
  raptor_can_rxmsg4/2 -> Bus Creator4/2  "STMM_counterMsg304"
  raptor_can_rxmsg4/1 -> Bus Creator4/1  "Age"
  raptor_can_rxmsg3/5 -> Bus Creator3/5  "STMM_segmentTemp111"
  raptor_can_rxmsg3/4 -> Bus Creator3/4  "STMM_segmentTemp110"
  raptor_can_rxmsg3/3 -> Bus Creator3/3  "STMM_segmentTemp109"
  raptor_can_rxmsg3/2 -> Bus Creator3/2  "STMM_counterMsg303"
  raptor_can_rxmsg3/1 -> Bus Creator3/1  "Age"
  raptor_can_rxmsg2/5 -> Bus Creator2/5  "STMM_segmentTemp108"
  raptor_can_rxmsg2/4 -> Bus Creator2/4  "STMM_segmentTemp107"
  raptor_can_rxmsg2/3 -> Bus Creator2/3  "STMM_segmentTemp106"
  raptor_can_rxmsg2/2 -> Bus Creator2/2  "STMM_counterMsg302"
  raptor_can_rxmsg2/1 -> Bus Creator2/1  "Age"
  raptor_can_rxmsg1/5 -> Bus Creator1/5  "STMM_segmentTemp105"
  raptor_can_rxmsg1/4 -> Bus Creator1/4  "STMM_segmentTemp104"
  raptor_can_rxmsg1/3 -> Bus Creator1/3  "STMM_segmentTemp103"
  raptor_can_rxmsg1/2 -> Bus Creator1/2  "STMM_counterMsg301"
  raptor_can_rxmsg1/1 -> Bus Creator1/1  "Age"
  raptor_can_rxmsg/5 -> Bus Creator/5  "STMM_segmentTemp102"
  raptor_can_rxmsg/4 -> Bus Creator/4  "STMM_segmentTemp101"
  raptor_can_rxmsg/3 -> Bus Creator/3  "STMM_segmentTemp100"
  raptor_can_rxmsg/2 -> Bus Creator/2  "STMM_counterMsg300"
  raptor_can_rxmsg/1 -> Bus Creator/1  "Age"
